simulink model "RefModel_Task"  (R2020a)
(part 3 of 5)

    |     RTInfo.Warning = ENUM_RTInfo_Warn.Warn_Path_Not_Valid;
    |     printComInfo('[System Warning] PathData Not Valid',tabspace1)
    | end
    | if ~IN_OnPlane.unlock
    | %     RTInfo.Warning = ENUM_RTInfo_Warn.Warn_SensorSystem_Not_Health;
    |     printComInfo('[System Warning] Not Unlock',tabspace1)
    | end
    | if isStallingForAWhile
    |     RTInfo.Warning = ENUM_RTInfo_Warn.Warn_Stalling;
    |     printComInfo('[System Warning] Stalling',tabspace1)
    | end
    | if ~isNaviFilterStart
    |     RTInfo.Warning = ENUM_RTInfo_Warn.Warn_FilterInit_Not_Complete;
    |     printComInfo('[System Warning] Filter Init Not Complete',tabspace1)
    | end
  function flag = isUavInFix2Rotor:
    | function flag = isUavInFix2Rotor
    | flag = false;
    | if PathModeOut.uavMode == ENUM_UAVMode.Fix2Rotor
    |     flag = true;
    | end
  function flag = isStallingForAWhile:
    | function flag = isStallingForAWhile
    | persistent lastNotStallTime stallTime0
    | if isempty(lastNotStallTime)
    |     lastNotStallTime = 0;
    |     stallTime0 = 0;
    | end
    | if ~isInStall
    |     lastNotStallTime = clock_sec; 
    | else
    |     stallTime0 = clock_sec;
    | end
    | flag = false;
    | if stallTime0 - lastNotStallTime > TaskParam.enterStallTimeSec
    |     flag = true;
    | end
  function flag = isUavInFix:
    | function flag = isUavInFix
    | flag = false;
    | if PathModeOut.uavMode == ENUM_UAVMode.Fix
    |     flag = true;
    | end
  function flag = isGetOutOfStall:
    | function flag = isGetOutOfStall
    | persistent lastStallTime notStallTime0
    | if isempty(lastStallTime)
    |     lastStallTime = 0;
    |     notStallTime0 = 0;
    | end
    | if ~isAttitudeStable_globalvar % 姿态不稳
    |     lastStallTime = clock_sec; 
    | else
    |     notStallTime0 = clock_sec;
    | end
    | flag = false;
    | if notStallTime0 - lastStallTime > 10 % 姿态稳定 10s 视为失速改出
    |     flag = true;
    | end
  function flag = willEnterManualMode:
    | function flag = willEnterManualMode
    | flag = false;
    | if ~isAutoMode_globalvar
    |     flag = true;
    | end
  function flag = willEnterAutoMode:
    | function flag = willEnterAutoMode
    | flag = false;
    | if isAutoMode_globalvar || (isNotInFense && PathModeOut.whereIsUAV == ENUM_Where.InTheAir) % && hasTaskStarted_globalbar
    |     flag = true;
    | end
  function setFlightModeInitState:
    | function setFlightModeInitState
    | % 飞机在地面的初始状态
    | PathModeOut.whereIsUAV = ENUM_Where.OnGround;  % 在地面
    | PathModeOut.uavMode = ENUM_UAVMode.Rotor;  % 旋翼
  function du_AUTO_TASK_func:
    | function du_AUTO_TASK_func
    | if isUavInRotor
    |     % dz: 固定翼航线模式下表示侧偏距，旋翼模式表示到目标点/悬停点的距离
    |     PathModeOut.distToGo = distOfTwoLL(PathModeOut.turnCenterLL(1:2),...
    |         ComFlightOut.curLLA(1:2));
    |     if all(PathModeOut.turnCenterLL(1:2)== 0) || all(ComFlightOut.curLLA(1:2)== 0)
    |         PathModeOut.distToGo = 0;
    |     end
    | end
  function sendEventWhileEnterAuto:
    | function sendEventWhileEnterAuto
    | PathModeOut.typeAutoMode = ENUM_AutoModeType.NotAutoMode; % 默认是非自动全剖面飞行
    | switch PathModeOut.whereIsUAV
    |     case ENUM_Where.OnGround % 在地面
    |         RTInfo.Task = ENUM_RTInfo_Task.Switch_AutoMode_sendEventWhileSwitchToAuto_OnGround; % 更新RT信息
    |         PathModeOut.typeAutoMode = ENUM_AutoModeType.ManualToAuto; % 只有在地面触发
    |         send(manual_groundStandBy,FLIGHTMODE.AUTO_TASK);
    |     case ENUM_Where.InTheAir % 在空中
    |         RTInfo.Task = ENUM_RTInfo_Task.Switch_AutoMode_sendEventWhileSwitchToAuto_InTheAir; % 更新RT信息
    |         isEverythingOk = ~isNotInFense && ... % 在区域内 且
    |                 PathModeOut.comStatus == ENUM_ComStatus.ComNormal; % 通信正常
    |         if isEverythingOk
    |             PathModeOut.typeAutoMode = ENUM_AutoModeType.ManualToAuto;
    |             if PathModeOut.uavMode == ENUM_UAVMode.Rotor % 空中/旋翼, 进入空中绕飞待命模式
    |                 RTInfo.Task = ENUM_RTInfo_Task.Switch_AutoMode_sendEventWhileSwitchToAuto_InTheAir_If_Rotor; % 更新RT信息
    |                 send(manual_hoverAdjust,FLIGHTMODE.AUTO_TASK);
    |             elseif PathModeOut.uavMode == ENUM_UAVMode.Fix % 空中/固定翼, 进入悬停调整模式
    |                 RTInfo.Task = ENUM_RTInfo_Task.Switch_AutoMode_sendEventWhileSwitchToAuto_InTheAir_If_Fix; % 更新RT信息
    |                 send(manual_airStandBy,FLIGHTMODE.AUTO_TASK);
    |             else
    |                 % 未处理状态
    |                 send(manual_hoverAdjust,FLIGHTMODE.AUTO_TASK);
    |                 RTInfo.Task = ENUM_RTInfo_Task.NotDefined_Fcn_sendEventWhileSwitchToAuto_If; % 更新RT信息
    |                 printComInfo('[Error] UAV is not Fix or Rotor when switch to AUTO_TASK',0)
    |             end
    |         else % 不在篱笆内 或 通信中断
    |             RTInfo.Task = ENUM_RTInfo_Task.Switch_AutoMode_sendEventWhileSwitchToAuto_InTheAir_NotInFense; % 更新RT信息
    |             printComInfo('[Info] Switch to AUTO_TASK, then enter GoHome mode',0)
    |             PathModeOut.typeAutoMode = ENUM_AutoModeType.SuspendTaskToHome;
    |             send(event_goHome_NotInFense,FLIGHTMODE.AUTO_TASK);
    |         end
    |     otherwise
    |         % 未处理状态
    |         RTInfo.Task = ENUM_RTInfo_Task.NotDefined_Fcn_sendEventWhileSwitchToAuto_Switch; % 更新RT信息
    |         printComInfo('[Error] UAV is not OnGround or InTheAir when switch to AUTO_TASK',0)
    | end
  function flag = isAllowedToEnterThisMode(mode):
    | function flag = isAllowedToEnterThisMode(mode)
    | flag = false;
    | tabspace1 = 2;
    | tabspace2 = 3;
    | % if isUavInRotor2Fix % 应对当前模式为 Rotor2Fix 或 Fix2Rotor
    | %     PathModeOut.uavMode = ENUM_UAVMode.Fix;
    | % elseif isUavInFix2Rotor
    | %     PathModeOut.uavMode = ENUM_UAVMode.Rotor;
    | % end
    | switch mode
    |     case ENUM_FlightTaskMode.TakeOffMode
    |         flag = isAllowedToTakeOff;
    |         if ~flag
    |             RTInfo.Task = ENUM_RTInfo_Task.SendEvent_TakeOff_ButNotAllowed; % 更新RT信息
    |             updateLogDataBuffer(ENUM_TaskLogBlockName.TASKLOG_FlightMode,RTInfo.Task,'write'); % 更新log缓存
    |             printComInfo('isAllowedToEnterThisMode() Switch TakeOffMode No',tabspace1)
    |             if not(isAllowedToTakeOff)
    |                 printComInfo('Not Allowed To TakeOff',tabspace2)
    |             end
    |             if ~isOnGround
    |                 printComInfo('Is Not OnGround',tabspace2)
    |             end
    |             if ~isUavInRotor
    |                 printComInfo('Is Not Rotor',tabspace2)
    |             end
    |             if not(BatteryOut.batteryStatus == ENUM_BatteryStatus.BatteryNormal)
    |                 printComInfo('BatteryLife Is Not Normal',tabspace2)
    |             end
    |         else
    |             printComInfo('isAllowedToEnterThisMode() Switch TakeOffMode Yes',tabspace1)
    |         end
    |     case ENUM_FlightTaskMode.HoverAdjustMode
    |         flag = isInTheAir && isUavInRotor && ...
    |             PathModeOut.flightTaskMode ~= ENUM_FlightTaskMode.Rotor2Fix_Mode && ...
    |             PathModeOut.flightTaskMode ~= ENUM_FlightTaskMode.Fix2Rotor_Mode;    
    |         if ~flag
    |             RTInfo.Task = ENUM_RTInfo_Task.SendEvent_HoverAdjust_ButNotAllowed; % 更新RT信息
    |             printComInfo('isAllowedToEnterThisMode() Switch HoverAdjustMode No',tabspace1)
    |             if not(isAllowedToAutoFlight)
    |                 printComInfo('Not Allowed To AutoFlight',tabspace2)
    |             end
    |             if ~isInTheAir
    |                 printComInfo('Is Not InTheAir',tabspace2)
    |             end
    |             if ~isUavInRotor
    |                 printComInfo('Is Not Rotor',tabspace2)
    |             end
    |         else
    |             printComInfo('isAllowedToEnterThisMode() Switch HoverAdjustMode Yes',tabspace1)            
    |         end
    |     case ENUM_FlightTaskMode.Rotor2Fix_Mode
    |         flag = isAllowedToAutoFlight && isInTheAir && isUavInRotor;
    |         if ~flag
    |             RTInfo.Task = ENUM_RTInfo_Task.SendEvent_Rotor2Fix_ButNotAllowed; % 更新RT信息
    |             printComInfo('isAllowedToEnterThisMode() Switch Rotor2Fix_Mode No',tabspace1)
    |             if not(isAllowedToAutoFlight)
    |                 printComInfo('Not Allowed To AutoFlight',tabspace2)
    |             end
    |             if ~isInTheAir
    |                 printComInfo('Is Not InTheAir',tabspace2)
    |             end
    |             if ~isUavInRotor
    |                 printComInfo('Is Not Rotor',tabspace2)
    |             end
    |         else
    |             printComInfo('isAllowedToEnterThisMode() Switch Rotor2Fix_Mode Yes',tabspace1)                  
    |         end
    |     case ENUM_FlightTaskMode.HoverUpMode
    |         flag = isAllowedToAutoFlight && isInTheAir && isUavInFix;
    |         if ~flag
    |             RTInfo.Task = ENUM_RTInfo_Task.SendEvent_HoverUp_ButNotAllowed; % 更新RT信息
    |             printComInfo('isAllowedToEnterThisMode() Switch HoverUpMode No',tabspace1)
    |             if not(isAllowedToAutoFlight)
    |                 printComInfo('Not Allowed To AutoFlight',tabspace2)
    |             end
    |             if ~isInTheAir
    |                 printComInfo('Is Not InTheAir',tabspace2)
    |             end
    |             if ~isUavInFix
    |                 printComInfo('Is Not Fix',tabspace2)
    |             end
    |         else
    |             printComInfo('isAllowedToEnterThisMode() Switch HoverUpMode Yes',tabspace1)                  
    |         end
    |     case ENUM_FlightTaskMode.PathFollowMode
    |         flag = isAllowedToAutoFlight && isInTheAir && isUavInFix;
    |         if ~flag
    |             RTInfo.Task = ENUM_RTInfo_Task.SendEvent_PathFollow_ButNotAllowed; % 更新RT信息
    |             printComInfo('isAllowedToEnterThisMode() Switch PathFollowMode No',tabspace1)
    |             if not(isAllowedToAutoFlight)
    |                 printComInfo('Not Allowed To AutoFlight',tabspace2)
    |             end
    |             if ~isInTheAir
    |                 printComInfo('Is Not InTheAir',tabspace2)
    |             end
    |             if ~isUavInFix
    |                 printComInfo('Is Not Fix',tabspace2)
    |             end               
    |         else
    |             printComInfo('isAllowedToEnterThisMode() Switch PathFollowMode Yes',tabspace1)                  
    |         end
    |     case ENUM_FlightTaskMode.GoHomeMode 
    |         flag = isInTheAir && (isUavInRotor || isUavInFix);
    |         if ~flag
    |             RTInfo.Task = ENUM_RTInfo_Task.SendEvent_GoHomeMode_ButNotAllowed; % 更新RT信息
    |             printComInfo('isAllowedToEnterThisMode() Switch GoHomeMode No',tabspace1)
    |             if not(isAllowedToAutoFlight)
    |                 printComInfo('Not Allowed To AutoFlight',tabspace2)
    |             end
    |             if ~isInTheAir
    |                 printComInfo('Is Not InTheAir',tabspace2)
    |             end
    |             if not(isUavInRotor || isUavInFix)
    |                 printComInfo('Is Not Fix or Rotor',tabspace2)
    |             end                  
    |         else
    |             printComInfo('isAllowedToEnterThisMode() Switch GoHomeMode Yes',tabspace1)                  
    |         end
    |     case ENUM_FlightTaskMode.HoverDownMode
    |         flag = isInTheAir && isUavInFix;
    |         if ~flag
    |             RTInfo.Task = ENUM_RTInfo_Task.SendEvent_HoverDown_ButNotAllowed; % 更新RT信息
    |             printComInfo('isAllowedToEnterThisMode() Switch HoverDownMode No',tabspace1)
    |             if not(isAllowedToAutoFlight)
    |                 printComInfo('Not Allowed To AutoFlight',tabspace2)
    |             end
    |             if ~isInTheAir
    |                 printComInfo('Is Not InTheAir',tabspace2)
    |             end
    |             if ~isUavInFix
    |                 printComInfo('Is Not Fix',tabspace2)
    |             end               
    |         else
    |             printComInfo('isAllowedToEnterThisMode() Switch HoverDownMode Yes',tabspace1)                  
    |         end
    |     case ENUM_FlightTaskMode.Fix2Rotor_Mode
    |         flag = isInTheAir && (isUavInFix || isUavInRotor2Fix);
    |         if ~flag
    |             RTInfo.Task = ENUM_RTInfo_Task.SendEvent_Fix2Rotor_ButNotAllowed; % 更新RT信息
    |             printComInfo('isAllowedToEnterThisMode() Switch Fix2Rotor_Mode No',tabspace1)
    |             if ~isInTheAir
    |                 printComInfo('Is Not InTheAir',tabspace2)
    |             end
    |             if ~isUavInFix
    |                 printComInfo('Is Not Fix',tabspace2)
    |             end                     
    |         else
    |             printComInfo('isAllowedToEnterThisMode() Switch Fix2Rotor_Mode Yes',tabspace1)                  
    |         end
    |     case ENUM_FlightTaskMode.LandMode
    |         flag = isInTheAir && isUavInRotor;
    |         if ~flag
    |             RTInfo.Task = ENUM_RTInfo_Task.SendEvent_Land_ButNotAllowed; % 更新RT信息
    |             printComInfo('isAllowedToEnterThisMode() Switch LandMode No',tabspace1)
    |             if not(isAllowedToAutoFlight)
    |                 printComInfo('Not Allowed To AutoFlight',tabspace2)
    |             end
    |             if ~isInTheAir
    |                 printComInfo('Is Not InTheAir',tabspace2)
    |             end
    |             if ~isUavInRotor
    |                 printComInfo('Is Not Rotor',tabspace2)
    |             end                 
    |         else
    |             printComInfo('isAllowedToEnterThisMode() Switch LandMode Yes',tabspace1)                  
    |         end
    |     case ENUM_FlightTaskMode.AirStandByMode
    |         flag = isInTheAir && canEnterAirStandByMode;
    |         if ~flag
    |             RTInfo.Task = ENUM_RTInfo_Task.SendEvent_AirStandBy_ButNotAllowed; % 更新RT信息
    |             printComInfo('isAllowedToEnterThisMode() Switch AirStandByMode No',tabspace1)
    |             if not(isAllowedToAutoFlight)
    |                 printComInfo('Not Allowed To AutoFlight',tabspace2)
    |             end
    |             if ~isInTheAir
    |                 printComInfo('Is Not InTheAir',tabspace2)
    |             end
    |             if not(canEnterAirStandByMode)
    |                 printComInfo('Can Not EnterAirStandByMode',tabspace2)
    |             end               
    |         else
    |             printComInfo('isAllowedToEnterThisMode() Switch AirStandByMode Yes',tabspace1)                  
    |         end
    |     otherwise
    |         RTInfo.Task = ENUM_RTInfo_Task.NotDefined_Fcn_isAllowedToEnterThisMode; % 更新RT信息
    |         printComInfo('isAllowedToEnterThisMode() Switch Otherwise',0)
    | end
  function dist = calDradiusWhileTurn(Rtarget,LL1,LL2):
    | function dist = calDradiusWhileTurn(Rtarget,LL1,LL2)
    | pos = lla2ned([LL1;0]', LL2');
    | Rnow = norm(pos(1:2));
    | dist = Rtarget - Rnow;
  function flag = isReadyToGo:
    | function flag = isReadyToGo
    | flag = 1;
    | if flag == 1 && isAttitudeStable_globalvar && isDebugInfoToShow
    |     fprintf('\t\t\t time %.2f [sec]: Ready To Go!\n',clock_sec);
    | end
  function flag = hasReachHeight(heightErr):
    | function flag = hasReachHeight(heightErr)
    | flag = false;
    | % heightErr = abs(ComFlightOut.curLLA(3)-PathModeOut.heightCmd);
    | if ComFlightOut.curLLA(3)>PathModeOut.heightCmd-heightErr
    |     flag = true;
    |     if isDebugInfoToShow
    | %         fprintf('\t\t\t time %.2f [sec]: Reach The Expected Hover Height %.0f [m]!\n',clock_sec,PathModeOut.heightCmd);
    |     end
    | end
  function headingCmd = calHeadingCmd(uavLLA_in,targetLLA_in):
    | function headingCmd = calHeadingCmd(uavLLA_in,targetLLA_in)
    | % 计算应飞航向
    | % pUAV: 无人机当前位置
    | % pointXY: 当前航线终点
    | % headingCmd: 应飞航向 (-pi,pi]
    | cPos = lla2ned(uavLLA_in, uavLLA_in(1:2));
    | target = lla2ned(targetLLA_in, uavLLA_in(1:2));
    | % 矢量
    | vec = target - cPos;
    | % 计算应飞航向
    | headingCmd = atan2(vec(2),vec(1));
  function flag = hasReachLatLon_assign(posErr):
    | function flag = hasReachLatLon_assign(posErr)
    | flag = false;
    | dLat = PathModeOut.turnCenterLL(1)- ComFlightOut.curLLA(1);
    | dLon = PathModeOut.turnCenterLL(2)- ComFlightOut.curLLA(2);
    | deg2m = 111e3;
    | dPn = dLat*deg2m;
    | dPe = dLon*deg2m*cos(ComFlightOut.curLLA(1)*pi/180);
    | dist = norm([dPn,dPe]);
    | if dist < posErr
    |     flag = true;
    | end
  function flag = isHeadingOk:
    | function flag = isHeadingOk
    | flag = false;
    | errAngle = angdiff(ComFlightOut.curEuler(1),headingCmd);
    | if abs(errAngle)<20*pi/180
    |     flag = true;
    |     printDebugInfo('AirStandBy','Already Heading To Target',2)
    | end
  function flag = isReadyToGo:
    | function flag = isReadyToGo
    | % TODO
    | flag = 1;
    | if flag == 1
    |     if isDebugInfoToShow
    |         fprintf('\t\t\t time %.2f [sec]: [HoverAdjust Mode] Ready To Go!\n',clock_sec);
    |     end
    | end
  function flag = hasReachHeight:
    | function flag = hasReachHeight
    | flag = false;
    | heightErr = abs(ComFlightOut.curLLA(3)-PathModeOut.heightCmd);
    | if ComFlightOut.curLLA(3) > PathModeOut.heightCmd - 2
    |     flag = true;
    | %     RTInfo.Task = ENUM_RTInfo_Task.If_AutoMode_HoverAdjust_ReachHeight_Yes; % 更新RT信息
    | %     if isDebugInfoToShow
    | %         fprintf('\t\t\t time %.2f [sec]: Reach The Expected Hover Height %.0f [m]!\n',clock_sec,PathModeOut.heightCmd);
    | %     end
    | end
  function flag = hasMatchAllConditons:
    | function flag = hasMatchAllConditons
    | persistent flagPre
    | if isempty(flagPre)
    |     flagPre = false;
    | end
    | flag = false;
    | if hasReachHeight && hasReachLatLon && isAttitudeStable_globalvar
    |     flag = true;
    |     RTInfo.Task = ENUM_RTInfo_Task.If_AutoMode_HoverAdjust_ReachHeightAndLevelPoint_Yes; % 更新RT信息
    |     if isDebugInfoToShow && flag ~= flagPre
    |         fprintf('\t\t\t time %.2f [sec]: Reach The Expected Hover Height %.0f [m] and Level Point (%.6f, %.6f)!\n',...
    |             clock_sec,PathModeOut.heightCmd,PathModeOut.turnCenterLL(1),PathModeOut.turnCenterLL(2));
    |     end
    | end
    | flagPre = flag;
  function flag = hasReachLatLon:
    | function flag = hasReachLatLon
    | flag = false;
    | dLat = PathModeOut.turnCenterLL(1)- ComFlightOut.curLLA(1);
    | dLon = PathModeOut.turnCenterLL(2)- ComFlightOut.curLLA(2);
    | deg2m = 111e3;
    | dPn = dLat*deg2m;
    | dPe = dLon*deg2m*cos(ComFlightOut.curLLA(1)*pi/180);
    | dist = norm([dPn,dPe]);
    | if dist < 3
    |     flag = true;
    | end
  function en_func:
    | function en_func
    | RTInfo.Task = ENUM_RTInfo_Task.Enter_AutoMode_HoverAdjust_Init; % 更新RT信息
    | updateLogDataBuffer(ENUM_TaskLogBlockName.TASKLOG_FlightMode,RTInfo.Task,'write'); % 更新log缓存
    | PathModeOut.uavMode = TaskParam.uavMode_InHoverAdjustMode;
    | PathModeOut.flightTaskMode = ENUM_FlightTaskMode.HoverAdjustMode;
    | PathModeOut.flightControlMode = ENUM_FlightControlMode.SpotHoverMode;
    | % 需计算指令： 高度 航向
    | tempIdx = idxStartPathPoint;
    | if isPathDataValid && PathModeOut.typeAutoMode == ENUM_AutoModeType.AutoProfile
    |     % 自动任务模式下
    |     printDebugInfo('HoverAdjust','Init AutoProfile Yes')
    |     RTInfo.Task = ENUM_RTInfo_Task.If_AutoMode_HoverAdjust_Init_AutoProfile_Yes; % 更新RT信息
    |     updateLogDataBuffer(ENUM_TaskLogBlockName.TASKLOG_FlightMode,RTInfo.Task,'write'); % 更新log缓存
    |     % 高度指令与前一模式相同
    |     if headingMode == 1
    |         targetLLA = double([IN_MAV.mavlink_mission_item_def(tempIdx).x,...
    |             IN_MAV.mavlink_mission_item_def(tempIdx).y, IN_MAV.mavlink_mission_item_def(tempIdx).z]);
    |         PathModeOut.headingCmd = calHeadingCmd(...
    |             ComFlightOut.curLLA,  targetLLA);
    |     else
    |         % 捕获当前航向
    |         PathModeOut.headingCmd = double(ComFlightOut.curEuler(1));
    |     end
    | else
    |     printDebugInfo('HoverAdjust','Init AutoProfile No')
    |     RTInfo.Task = ENUM_RTInfo_Task.If_AutoMode_HoverAdjust_Init_AutoProfile_No; % 更新RT信息
    |     updateLogDataBuffer(ENUM_TaskLogBlockName.TASKLOG_FlightMode,RTInfo.Task,'write'); % 更新log缓存
    |     % 捕获当前航向
    |     PathModeOut.headingCmd = double(ComFlightOut.curEuler(1));
    |     % 捕获当前高度
    |     PathModeOut.heightCmd = double(ComFlightOut.curLLA(3));
    | end
    | PathModeOut.groundspeedCmd = TaskParam.cruiseSpeed_rotorMode;
    | % 设置侧偏距为0
    | PathModeOut.dz = 0;
    | % 设置预置滚转
    | PathModeOut.rollCmd = 0;
    | % 悬停位置
    | PathModeOut.turnCenterLL = ComFlightOut.curLLA(1:2);
    | % 最大爬升率
    | PathModeOut.maxClimbSpeed = TaskParam.maxClimbSpeed_normal_TakeOffandLand;
  function responseManualMove:
    | function responseManualMove
    | persistent nFront nBack nRight nLeft
    | if isempty(nFront)
    | %     nFront = -99;
    | %     nBack = -99;
    | %     nRight = -99;
    | %     nLeft = -99;
    |     nFront = IN_MAV.mavlink_msg_arrowkey.nFront;
    |     nBack = IN_MAV.mavlink_msg_arrowkey.nBack;
    |     nRight = IN_MAV.mavlink_msg_arrowkey.nRight;
    |     nLeft = IN_MAV.mavlink_msg_arrowkey.nLeft;    
    | end
    | %%
    | nFront_cur = IN_MAV.mavlink_msg_arrowkey.nFront;
    | nBack_cur = IN_MAV.mavlink_msg_arrowkey.nBack;
    | nRight_cur = IN_MAV.mavlink_msg_arrowkey.nRight;
    | nLeft_cur = IN_MAV.mavlink_msg_arrowkey.nLeft;
    | distFront = IN_MAV.mavlink_msg_arrowkey.distFront;
    | distRight = IN_MAV.mavlink_msg_arrowkey.distRight;
    | distBack = IN_MAV.mavlink_msg_arrowkey.distBack;
    | distLeft = IN_MAV.mavlink_msg_arrowkey.distLeft;
    | curLat = ComFlightOut.curLLA(1);
    | %%
    | dP_lat = 0;
    | dP_lon = 0;
    | heading = ComFlightOut.curEuler(1);
    | if nFront ~= nFront_cur
    |     angle = heading + 0;
    |     dP_lat = dP_lat + distFront*cos(angle);
    |     dP_lon = dP_lon + distFront*sin(angle);
    |     RTInfo.Task = ENUM_RTInfo_Task.Event_GSKeyMove_North;
    |     printComInfo('Key Move: Front %.0fm',1,distFront);
    | end
    | if nBack ~= nBack_cur
    |     angle = heading + pi;
    |     dP_lat = dP_lat + distBack*cos(angle);
    |     dP_lon = dP_lon + distBack*sin(angle);
    |     RTInfo.Task = ENUM_RTInfo_Task.Event_GSKeyMove_South;
    |     printComInfo('Key Move: Back %.0fm',1,distBack);
    | end
    | if nRight ~= nRight_cur
    |     angle = heading + pi/2;
    |     dP_lat = dP_lat + distRight*cos(angle);
    |     dP_lon = dP_lon + distRight*sin(angle);
    |     RTInfo.Task = ENUM_RTInfo_Task.Event_GSKeyMove_East;
    |     printComInfo('Key Move: Right %.0fm',1,distRight);
    | end
    | if nLeft ~= nLeft_cur
    |     angle = heading + 3/2*pi;
    |     dP_lat = dP_lat + distLeft*cos(angle);
    |     dP_lon = dP_lon + distLeft*sin(angle);
    |     RTInfo.Task = ENUM_RTInfo_Task.Event_GSKeyMove_West;
    |     printComInfo('Key Move: Left %.0fm',1,distLeft);
    | end
    | nFront = IN_MAV.mavlink_msg_arrowkey.nFront;
    | nBack = IN_MAV.mavlink_msg_arrowkey.nBack;
    | nRight = IN_MAV.mavlink_msg_arrowkey.nRight;
    | nLeft = IN_MAV.mavlink_msg_arrowkey.nLeft;
    | 
    | dlat_deg = m2lat(dP_lat);
    | dlon_deg = m2lon(dP_lon,curLat);
    | if dlat_deg ~= 0 || dlon_deg ~= 0
    |     PathModeOut.turnCenterLL = PathModeOut.turnCenterLL + [dlat_deg,dlon_deg];
    |     ComFlightOut.curHomeLLA(1:2) = PathModeOut.turnCenterLL;
    |     RTInfo.Task = ENUM_RTInfo_Task.TaskLog_Input_HomeChange_KeyBoard;% 更新RTInfo Task
    |     updateLogDataBuffer(ENUM_TaskLogBlockName.TASKLOG_ParserInput,RTInfo.Task,'write'); % 更新log缓存
    | end
  function en_func:
    | function en_func
    | printDebugInfo('HoverAdjust','Doing')
    | RTInfo.Task = ENUM_RTInfo_Task.Enter_AutoMode_HoverAdjust_Doing; % 更新RT信息
    | updateLogDataBuffer(ENUM_TaskLogBlockName.TASKLOG_FlightMode,RTInfo.Task,'write'); % 更新log缓存
    | switch PathModeOut.typeAutoMode
    |     case ENUM_AutoModeType.SuspendTaskToHomeThenLand
    |         printDebugInfo('HoverAdjust','Switch SuspendTaskToHomeThenLand')
    |         RTInfo.Task = ENUM_RTInfo_Task.Switch_AutoMode_HoverAdjust_Doing_SuspendTaskToHome; % 更新RT信息
    |         updateLogDataBuffer(ENUM_TaskLogBlockName.TASKLOG_FlightMode,RTInfo.Task,'write'); % 更新log缓存
    |         PathModeOut.turnCenterLL = ComFlightOut.curHomeLLA(1:2);
    |     case  ENUM_AutoModeType.SuspendTaskToLand
    |         printDebugInfo('HoverAdjust','Switch SuspendTaskToLand')
    |         RTInfo.Task = ENUM_RTInfo_Task.Switch_AutoMode_HoverAdjust_Doing_SuspendTaskToLand; % 更新RT信息
    |         updateLogDataBuffer(ENUM_TaskLogBlockName.TASKLOG_FlightMode,RTInfo.Task,'write'); % 更新log缓存
    |         if landPosMode == ENUM_LandMode.HomeVTL
    |             PathModeOut.turnCenterLL = ComFlightOut.curHomeLLA(1:2);
    |         else
    |             PathModeOut.turnCenterLL = ComFlightOut.curLLA(1:2);
    |         end
    |     case ENUM_AutoModeType.SuspendTaskToHome
    |         printDebugInfo('HoverAdjust','Switch SuspendTaskToHome')
    |         RTInfo.Task = ENUM_RTInfo_Task.Switch_AutoMode_HoverAdjust_Doing_SuspendTaskToHome; % 更新RT信息
    |         updateLogDataBuffer(ENUM_TaskLogBlockName.TASKLOG_FlightMode,RTInfo.Task,'write'); % 更新log缓存
    |         PathModeOut.turnCenterLL = ComFlightOut.curLLA(1:2);
    |     case ENUM_AutoModeType.Fix2Rotor2HoverAdjust
    |         printDebugInfo('HoverAdjust','Switch Fix2Rotor2HoverAdjust')
    |         RTInfo.Task = ENUM_RTInfo_Task.Switch_AutoMode_HoverAdjust_Doing_Fix2Rotor2HoverAdjust; % 更新RT信息
    |         updateLogDataBuffer(ENUM_TaskLogBlockName.TASKLOG_FlightMode,RTInfo.Task,'write'); % 更新log缓存
    |         PathModeOut.turnCenterLL = ComFlightOut.curLLA(1:2);
    |     case ENUM_AutoModeType.AutoProfile
    |         printDebugInfo('HoverAdjust','Switch AutoProfile')
    |         RTInfo.Task = ENUM_RTInfo_Task.Switch_AutoMode_HoverAdjust_Doing_AutoProfile; % 更新RT信息
    |         updateLogDataBuffer(ENUM_TaskLogBlockName.TASKLOG_FlightMode,RTInfo.Task,'write'); % 更新log缓存
    |         if nextMode == ENUM_FlightTaskMode.LandMode
    |             PathModeOut.turnCenterLL = ComFlightOut.curHomeLLA(1:2);
    |         end
    |     case ENUM_AutoModeType.PauseInAir
    |         RTInfo.Task = ENUM_RTInfo_Task.Switch_AutoMode_HoverAdjust_Doing_PauseInAir; % 更新RT信息
    |         updateLogDataBuffer(ENUM_TaskLogBlockName.TASKLOG_FlightMode,RTInfo.Task,'write'); % 更新log缓存        
    |         PathModeOut.typeAutoMode = typeAutoModePre;
    |         send(event_gotoWaitForContinue,FLIGHTMODE.AUTO_TASK)
    |     case ENUM_AutoModeType.Fix2Rotor2Home2Land
    |         printDebugInfo('HoverAdjust','Switch Fix2Rotor2Home2Land')
    |         RTInfo.Task = ENUM_RTInfo_Task.Switch_AutoMode_HoverAdjust_Doing_PauseInAir; % 更新RT信息
    |         updateLogDataBuffer(ENUM_TaskLogBlockName.TASKLOG_FlightMode,RTInfo.Task,'write'); % 更新log缓存              
    |         PathModeOut.turnCenterLL = ComFlightOut.curHomeLLA(1:2);
    |     otherwise
    |         % printDebugInfo('HoverAdjust','Switch Otherwise')
    |         RTInfo.Task = ENUM_RTInfo_Task.Switch_AutoMode_HoverAdjust_Doing_Otherwise; % 更新RT信息
    |         updateLogDataBuffer(ENUM_TaskLogBlockName.TASKLOG_FlightMode,RTInfo.Task,'write'); % 更新log缓存             
    |         RTInfo.Task = ENUM_RTInfo_Task.NotDefined_State_HoverAdjust_Doing_Switch; % 更新RT信息
    | end
  function dHeading = calHeadingErr(headingCmd,headingNow):
    | function dHeading = calHeadingErr(headingCmd,headingNow)
    | % 计算飞机当前航向偏差
    | % headingCmd: 指令航向 rad
    | % headingNow：当前航向 rad
    | % dHeading: 航向差 rad
    | headingNow = rem(headingNow,2*pi);
    | headingCmd = rem(headingCmd,2*pi);
    | sub = zeros(3,1);
    | psi_d_possible = zeros(3,1);
    | psi_d_possible(1) = headingCmd;
    | psi_d_possible(2) = headingCmd-2*pi;
    | psi_d_possible(3) = headingCmd+2*pi;
    | sub(1) = psi_d_possible(1)-headingNow;
    | sub(2) = psi_d_possible(2)-headingNow;
    | sub(3) = psi_d_possible(3)-headingNow;
    | [~,ind] = min(abs(sub));
    | dHeading = sub(ind);
    | 
    | % % 测试用例
    | % if 0
    | %     headingCmd = 181*pi/180;
    | %     headingNow = 179*pi/180;
    | %     dHeading = calHeadingErr(headingCmd,headingNow)*180/pi
    | %     
    | %     headingCmd = 361*pi/180;
    | %     headingNow = 359*pi/180;    
    | %     dHeading = calHeadingErr(headingCmd,headingNow)*180/pi    
    | %     
    | %     
    | %     headingCmd = -361*pi/180;
    | %     headingNow = -359*pi/180;
    | %     dHeading = calHeadingErr(headingCmd,headingNow)*180/pi  
    | %     
    | %     headingCmd = -1*pi/180;
    | %     headingNow = 0*pi/180;
    | %     dHeading = calHeadingErr(headingCmd,headingNow)*180/pi      
    | %     
    | %     headingCmd = -181*pi/180;
    | %     headingNow = 180*pi/180;
    | %     dHeading = calHeadingErr(headingCmd,headingNow)*180/pi    
    | % end
  function flag = hasReachExpectSpeed(airspeed_req,groundspeed_req):
    | function flag = hasReachExpectSpeed(airspeed_req,groundspeed_req)
    | flag = false;
    | if ComFlightOut.curGroundSpeed > groundspeed_req && ComFlightOut.curAirSpeed > airspeed_req
    |     flag = true;
    |     RTInfo.Task = ENUM_RTInfo_Task.If_AutoMode_Rotor2Fix_ReachSpeed_Yes; % 更新RT信息
    |     if isDebugInfoToShow
    | %         fprintf('\t\t\t time %.2f [sec]: Reach Expected Speed!\n',clock_sec);
    |     end
    | end
  function flag = calIfReachPoint_horizontal(uavLLA,point1LLA,point2LLA,In_AlgoParams):
    | function flag = calIfReachPoint_horizontal(uavLLA,point1LLA,point2LLA,In_AlgoParams)
    | % 判断是否到达目标点
    | % uavLLA: 当前位置
    | % point1LLA：航段起点位置
    | % point2LLA：航段终点位置
    | % In_AlgoParams: 参数
    | pUAV = lla2ned(uavLLA, uavLLA(1:2));
    | point1XY = lla2ned(point1LLA, uavLLA(1:2));
    | point2XY = lla2ned(point2LLA, uavLLA(1:2));
    | pUAV(3) = 0;
    | point1XY(3) = 0;
    | point2XY(3) = 0;
    | mode = In_AlgoParams.reachDetermineMode;
    | flag = false;
    | switch mode
    |     case 0 %
    |         reachFlag_point = calPointModeFlag(pUAV,point2XY,In_AlgoParams.reachFlag_point_dist);
    |         flag = reachFlag_point;
    |     case 1 %
    |         reachFlag_line = calLineModeFlag(pUAV,point2XY,point1XY,In_AlgoParams.reachFlag_line_dist);
    |         flag = reachFlag_line;
    |     case 2 %
    |         reachFlag_point = calPointModeFlag(pUAV,point2XY,In_AlgoParams.reachFlag_point_dist);
    |         reachFlag_line = calLineModeFlag(pUAV,point2XY,point1XY,In_AlgoParams.reachFlag_line_dist);
    |         flag = reachFlag_point | reachFlag_line;
    |     otherwise
    |         RTInfo.Task = ENUM_RTInfo_Task.NotDefined_Fcn_calIfReachPoint_Switch; % 更新RT信息
    |         error('Wrong set!')
    | end
    | if flag
    |      sl = 1; 
    | end
    | %% 点距判定
    | function reachFlag = calPointModeFlag(pUAV,point2XY,reachFlag_point_dist)
    | reachFlag = false;
    | dist = norm(pUAV-point2XY);
    | if dist <= reachFlag_point_dist
    |     reachFlag = true;
    | end
    | % test
    | if dist < 10
    |     test = 1; 
    | end
    | %% 过线判定
    | function reachFlag = calLineModeFlag(pUAV,point2XY,point1XY,reachFlag_point_dist)
    | vec1 = pUAV-point1XY;
    | vec2 = point2XY-point1XY;
    | len1 = norm(vec1);
    | len2 = norm(vec2);
    | if len1 == 0 || len2 == 0
    |     angle = 0;
    | else
    |     % 真的出现过acos(1.000000000000001)产生复数
    |     temp = dot(vec1,vec2)/(len1*len2+eps);
    |     if temp > 1
    |         temp = 1;
    |     elseif temp < -1
    |         temp = -1;
    |     end
    |     angle = acos(temp);
    | end
    | reachFlag = false;
    | if (abs(len1*cos(angle)) > len2 - reachFlag_point_dist) && abs(angle)<pi/2
    |     reachFlag = true;
    | end
    | if len1*cos(angle)-len2 < 10
    |     test = 1; 
    | end
  function out = calEnterLLToFlyAround(centerLL,curLL,R):
    | function out = calEnterLLToFlyAround(centerLL,curLL,R)
    | % out;目标[纬度，精度]deg
    | % centerLL: home点[纬度，精度]deg，作为绕飞圆心
    | % curLL：起始位置
    | % R: 盘旋半径
    | [tangencyLL1,tangencyLL2] = findTangencyPointsLLA(centerLL,curLL,R);
    | mode = 'clockwise'; % anticlockwise
    | switch mode
    |     case 'clockwise'
    |         out = tangencyLL1;
    |     otherwise
    |         out = tangencyLL2;
    | end
  function en_func_HoverUp:
    | function en_func_HoverUp
    | % 需计算指令： 高度 速度 滚转角 转弯半径
    | tempIdx = 1; % 使用home点的高度  idxStartPathPoint;
    | PathModeOut.turnRadiusCmd = TaskParam.turnR;
    | if isPathDataValid && PathModeOut.typeAutoMode == ENUM_AutoModeType.AutoProfile
    |     RTInfo.Task = ENUM_RTInfo_Task.If_AutoMode_HoverUp_Init_AutoProfile_Yes; % 更新RT信息
    |     updateLogDataBuffer(ENUM_TaskLogBlockName.TASKLOG_FlightMode,RTInfo.Task,'write'); % 更新log缓存    
    |     PathModeOut.heightCmd = double(ComFlightOut.curLLA(3));
    |     PathModeOut.groundspeedCmd = TaskParam.cruiseSpeed_cruise;
    | else % 手动选择该模式
    |     % 捕获当前高度
    |     PathModeOut.heightCmd = double(ComFlightOut.curLLA(3));
    |     % 捕获当前速度,设定最小值
    |     PathModeOut.groundspeedCmd = max(TaskParam.cruiseSpeed_cruise,ComFlightOut.curGroundSpeed);
    | end
    | % PathModeOut.turnRadiusCmd = AlgoParams.turnR;
    | PathModeOut.rollCmd = ...
    |     atan(PathModeOut.groundspeedCmd^2/PathModeOut.turnRadiusCmd/9.8);
    | 
    | % 设置侧偏距为0
    | PathModeOut.dz = 0;
    | % 绕飞中心
    | if preTaskMode ~= ENUM_FlightTaskMode.HoverUpMode && ...
    |         preTaskMode ~= ENUM_FlightTaskMode.HoverDownMode
    |     % 距离home点距离
    |     distToHome = distOfTwoLL(ComFlightOut.curHomeLLA(1:2)', ComFlightOut.curLLA(1:2));
    |     if ~TaskParam.isHoverUpDownWithHome || distToHome > 300 
    |         % 当不以home点为盘旋中心，或当前位置距离home过远时
    |         [dLat,dLon] = calDLatLonOfRotateCenterFromCurPos(...
    |             ComFlightOut.curLLA(1:2)',ComFlightOut.curEuler(1),PathModeOut.turnRadiusCmd,'right');
    |         PathModeOut.turnCenterLL =  ComFlightOut.curLLA(1:2) + [dLat,dLon];
    |     else
    |         % 以home点为盘旋中心，且home点在附近
    |         PathModeOut.turnCenterLL =  ComFlightOut.curHomeLLA(1:2);
    |         RTInfo.Task = ENUM_RTInfo_Task.If_AutoMode_INIT_CircleHome; % 更新RT信息
    |         updateLogDataBuffer(ENUM_TaskLogBlockName.TASKLOG_FlightMode,RTInfo.Task,'write'); % 更新log缓存
    |     end
    | else
    |     % 沿用HoverUpDown模式的，确保盘旋中心一致
    |     RTInfo.Task = ENUM_RTInfo_Task.HoverUp_INIT_ContinueHoverUpDown; % 更新RT信息
    |     updateLogDataBuffer(ENUM_TaskLogBlockName.TASKLOG_FlightMode,RTInfo.Task,'write'); % 更新log缓存
    | end
    | % 最大爬升率
    | PathModeOut.maxClimbSpeed = TaskParam.maxClimbSpeed_fixMode + 0.7;
  function flag = hasReachExpectedHeight:
    | function flag = hasReachExpectedHeight
    | flag = false;
    | if ComFlightOut.curLLA(3) > PathModeOut.heightCmd - 10
    |     flag = true;
    | %     RTInfo.Task = ENUM_RTInfo_Task.If_AutoMode_HoverUp_ReachHeight_Yes; % 更新RT信息
    | %     if isDebugInfoToShow
    | %         fprintf('\t\t\t time %.2f [sec]: Reach The Expected Hover Height %.0f [m]!\n',clock_sec,PathModeOut.heightCmd);
    | %     end
    | end
  function flag = hasReachExpectedHeightRange:
    | function flag = hasReachExpectedHeightRange
    | flag = false;
    | heightErr = abs(ComFlightOut.curLLA(3)-PathModeOut.heightCmd);
    | range = 10;
    | if heightErr < range
    |     flag = true;
    |     RTInfo.Task = ENUM_RTInfo_Task.If_AutoMode_HoverUp_ReachHeightRange_Yes; % 更新RT信息
    |     if isDebugInfoToShow
    |         fprintf('\t\t\t time %.2f [sec]: Reach The Expected Hover Height Range, Current Height is %.0f [m]!\n',clock_sec,PathModeOut.heightCmd);
    |     end
    | end
  function en_func_HoverUp_SingleMode:
    | function en_func_HoverUp_SingleMode
    | % 需计算指令： 高度 速度 滚转角 转弯半径
    | PathModeOut.turnRadiusCmd = TaskParam.turnR;
    | PathModeOut.heightCmd = double(ComFlightOut.curLLA(3)) + 100;
    | PathModeOut.groundspeedCmd = TaskParam.cruiseSpeed_cruise;
    | PathModeOut.rollCmd = ...
    |     atan(PathModeOut.groundspeedCmd^2/PathModeOut.turnRadiusCmd/9.8);
    | % 设置侧偏距为0
    | PathModeOut.dz = 0;
    | % 绕飞中心
    | [dLat,dLon] = calDLatLonOfRotateCenterFromCurPos(...
    |     ComFlightOut.curLLA(1:2)',ComFlightOut.curEuler(1),PathModeOut.turnRadiusCmd,'right');
    | PathModeOut.turnCenterLL =  ComFlightOut.curLLA(1:2) + [dLat,dLon];
    | % 最大爬升率
    | PathModeOut.maxClimbSpeed = TaskParam.maxClimbSpeed_fixMode;
  function updateTurnR_HoverUp:
    | function updateTurnR_HoverUp
    | % du_func_HoverUp_Doing
    | if ComFlightOut.curLLA(3) > TaskParam.beginHeight_expandRadiusInHoverUp
    |     % 半径扩张 (可以省电，但注意高度阈值的选择不易过低，否则有碰撞风险)
    |     dh = abs(ComFlightOut.curLLA(3) - TaskParam.beginHeight_expandRadiusInHoverUp);
    |     PathModeOut.turnRadiusCmd = TaskParam.turnR + TaskParam.k_expandRadiusInHoverUp*dh;
    |     PathModeOut.turnRadiusCmd = min(PathModeOut.turnRadiusCmd,TaskParam.maxRadiusInHoverUp);
    | end
    | PathModeOut.turnRadiusCmd_HoverUp = PathModeOut.turnRadiusCmd;
    | PathModeOut.dR_turn = calDradiusWhileTurn(PathModeOut.turnRadiusCmd,...
    |     ComFlightOut.curLLA(1:2)',PathModeOut.turnCenterLL);
  function flag = isHeadingToTarget:
    | function flag = isHeadingToTarget
    | flag = false;
    | tempIdx = idxStartPathPoint;
    | targetLLA = double([IN_MAV.mavlink_mission_item_def(tempIdx).x,...
    |     IN_MAV.mavlink_mission_item_def(tempIdx).y, IN_MAV.mavlink_mission_item_def(tempIdx).z]);
    | headingCmd = calHeadingCmd(ComFlightOut.curLLA,  targetLLA);
    | errAngle = angdiff(ComFlightOut.curEuler(1),headingCmd);
    | 
    | dist = distOfTwoLL(targetLLA(1:2),ComFlightOut.curLLA(1:2));
    | if abs(errAngle)<25*pi/180 || dist < 160
    |     flag = true;
    |     printDebugInfo('AirStandBy','Already Heading To Target',2)
    | end
  function record1(value):
    | function record1(value)
    | % record1
    | if value >= 90 && value < 120
    |     printDebugInfo('HoverUp','Expand R >= 90')
    | elseif value >= 120
    |     printDebugInfo('HoverUp','Expand R >= 120')
    | end
    | RTInfo.Task = ENUM_RTInfo_Task.HoverUp_Expand_R; % 更新RT信息
    | updateLogDataBuffer(ENUM_TaskLogBlockName.TASKLOG_FlightMode,RTInfo.Task,'write',[PathModeOut.turnRadiusCmd;0;0;0;0]); % 更新log缓存
  function SendEvent_autoGoToNextMode:
    | function SendEvent_autoGoToNextMode
    | send(auto_gotoNextMode,FLIGHTMODE.AUTO_TASK)
  function updateLLATaksInterrupt:
    | function updateLLATaksInterrupt
    | PathModeOut.LLATaskInterrupt = [...
    |     ComFlightOut.curLLA(1);...
    |     ComFlightOut.curLLA(2);...
    |     PathModeOut.heightCmd;];
    | PathModeOut.lastTargetPathPoint = PathModeOut.currentPointNum;
  function PathModeOut_out  = updatePathModeStruct(curLLA_param,startLLA_param,targetLLA_param,PathModeOut_in,mission_item_def_param):
    | function PathModeOut_out  = updatePathModeStruct(curLLA_param,startLLA_param,targetLLA_param,PathModeOut_in,mission_item_def_param)
    | % 更新航线模式的输出参数
    | PathModeOut_out = PathModeOut_in;
    | % 计算应飞航向
    | PathModeOut_out.headingCmd = calHeadingCmd(...
    |     curLLA_param,targetLLA_param);
    | % 计算剩余距离
    | PathModeOut_out.distToGo = calPointDist_horizontal(...
    |     curLLA_param, targetLLA_param);
    | % 计算侧偏距
    | PathModeOut_out.dz = calDz(ComFlightOut.curLLA,  ...
    |     startLLA_param,targetLLA_param);
    | % % 计算指令速度
    | % PathModeOut_out.groundspeedCmd = double(mission_item_def_param.param4);
    | % 计算转弯半径
    | % PathModeOut_out.turnRadiusCmd = 0;
    | % 计算指令高度
    | PathModeOut_out.heightCmd = double(mission_item_def_param.z);
  function updateTaskCompleteFlag:
    | function updateTaskCompleteFlag
    | PathModeOut.isTaskComplete = true;
  function dz = calDz(uavLLA,point1LLA,point2LLA):
    | function dz = calDz(uavLLA,point1LLA,point2LLA)
    | % 计算飞机当前位置偏离航线的距离
    | % pUAV: 无人机当前位置
    | % point0：当前航线起点
    | % point1: 当前航线终点
    | % dz: 侧偏距，从天顶俯视，飞机在航线右侧偏距为正
    | pUAV = lla2ned(uavLLA, point2LLA(1:2));
    | point1XY = lla2ned(point1LLA, point2LLA(1:2));
    | point2XY = lla2ned(point2LLA, point2LLA(1:2));
    | cPos = [pUAV(1:2),0];
    | point1 = [point1XY(1:2),0];
    | point2 = [point2XY(1:2),0];
    | % 矢量
    | vec1 = cPos-point1;
    | vec2 = point2-point1;
    | len1 = norm(vec1);
    | len2 = norm(vec2);
    | z = cross(vec1,vec2);
    | % 侧偏距
    | dz_sign = sign(z(3));
    | if len1 == 0 || len2 == 0
    |     sin_angle = 0;
    | else
    |     sin_angle = abs(norm(z)/len1/len2);
    | end
    | if abs(sin_angle) <= 1+1e-5
    |     sin_angle = min(max(sin_angle,-1),1);
    | elseif abs(sin_angle) > 1+1e-5
    |     sin_angle = sign(sin_angle);
    |     filename = 'calDz';
    |     error(['A error happened in ',filename]);
    | end
    | angle = asin(sin_angle);
    | dz = dz_sign*abs(sin(angle)*len1);
    | if isnan(dz)
    |     sl = 1;
    | end
    | %% 测试用例：
    | % if 0
    | %     num = 20;
    | %     point1XY = [-1,-1];
    | %     point2XY = [1,1];
    | %     figure(112)
    | %     plot(point1XY(1),point1XY(2),'ro');hold on;
    | %     plot(point2XY(1),point2XY(2),'bo');hold on;
    | %     plot([point1XY(1),point2XY(1)],[point1XY(2),point2XY(2)]);hold on;
    | %     grid on;
    | %     axis equal
    | %     xlim([-3,3])
    | %     ylim([-3,3])
    | %     pUAV = 1*randn(num,2);
    | %     for i = 1:num
    | %         dz(i) = calDz(pUAV(i,:),point1XY,point2XY);
    | %         plot(pUAV(i,1),pUAV(i,2),'k*');hold on;
    | %         text(pUAV(i,1)+0.2,pUAV(i,2)+0.2,[num2str(dz(i))]);hold on;
    | %     end
    | % end
  function flag = isNextTheLastPoint:
    | function flag = isNextTheLastPoint
    | % 计算有效航点数
    | flag = 0;
    | if PathModeOut.currentPointNum == PathModeOut.validPathNum
    |     flag = 1;
    | end
  function calTransitPoints:
    | function calTransitPoints
    | testflag = isAddTransitPoint && TaskParam.isInterpPathPoints;
    | % 判断当前航点和前置航点的距离
    | tempIdx = PathModeOut.prePointNum;
    | prePathLLA = double([IN_MAV.mavlink_mission_item_def(tempIdx).x,...
    |     IN_MAV.mavlink_mission_item_def(tempIdx).y, IN_MAV.mavlink_mission_item_def(tempIdx).z]);
    | tempIdx = PathModeOut.currentPointNum;
    | curPathLLA = double([IN_MAV.mavlink_mission_item_def(tempIdx).x,...
    |     IN_MAV.mavlink_mission_item_def(tempIdx).y, IN_MAV.mavlink_mission_item_def(tempIdx).z]);
    | distFromPrepathpointToCurpathpoint = distOfTwoLL(curPathLLA(1:2),prePathLLA(1:2));
    | if distFromPrepathpointToCurpathpoint < 1
    |     testflag = false;
    | end
    | % testflag = false;
    | if ~testflag
    |     % 航段起点
    |     tempIdx = PathModeOut.prePointNum;
    |     startLLA = double([IN_MAV.mavlink_mission_item_def(tempIdx).x,...
    |         IN_MAV.mavlink_mission_item_def(tempIdx).y, IN_MAV.mavlink_mission_item_def(tempIdx).z]);
    |     % 航段终点
    |     tempIdx = PathModeOut.currentPointNum;
    |     targetLLA = double([IN_MAV.mavlink_mission_item_def(tempIdx).x,...
    |         IN_MAV.mavlink_mission_item_def(tempIdx).y, IN_MAV.mavlink_mission_item_def(tempIdx).z]);
    |     
    |     temp_AlgoParams = TaskParam;
    |     kk = ComFlightOut.curGroundSpeed/(TaskParam.cruiseSpeed_cruise+eps);
    |     if isnan(kk)
    |         kk = 1;
    |     end
    |     kk = min(1.2,kk);
    |     kk = max(0.8,kk);
    |     temp_AlgoParams.reachFlag_point_dist = kk*temp_AlgoParams.reachFlag_point_dist; 
    |     arriveFlag = calIfReachPoint_horizontal(ComFlightOut.curLLA,  ...
    |         startLLA,  targetLLA,  temp_AlgoParams);
    | else
    |     minPoint0 = zeros(1,3);
    |     minPoint1 = zeros(1,3);
    |     minPoint2 = zeros(1,3);
    |     if PathModeOut.currentPointNum <= 2
    |         PathModeOut.currentPointNum = 3;
    |     end
    |     tempIdx = PathModeOut.currentPointNum-2;
    |     prepreLLA = double([IN_MAV.mavlink_mission_item_def(tempIdx).x,...
    |         IN_MAV.mavlink_mission_item_def(tempIdx).y, IN_MAV.mavlink_mission_item_def(tempIdx).z]);
    |     tempIdx = PathModeOut.currentPointNum-2;
    |     prepreLLA = double([IN_MAV.mavlink_mission_item_def(tempIdx).x,...
    |         IN_MAV.mavlink_mission_item_def(tempIdx).y, IN_MAV.mavlink_mission_item_def(tempIdx).z]);
    |     tempIdx = PathModeOut.currentPointNum-1;
    |     preLLA = double([IN_MAV.mavlink_mission_item_def(tempIdx).x,...
    |         IN_MAV.mavlink_mission_item_def(tempIdx).y, IN_MAV.mavlink_mission_item_def(tempIdx).z]);
    |     tempIdx = PathModeOut.currentPointNum;
    |     curLLA = double([IN_MAV.mavlink_mission_item_def(tempIdx).x,...
    |         IN_MAV.mavlink_mission_item_def(tempIdx).y, IN_MAV.mavlink_mission_item_def(tempIdx).z]);
    |     tempIdx = PathModeOut.currentPointNum+1;
    |     nextLLA = double([IN_MAV.mavlink_mission_item_def(tempIdx).x,...
    |         IN_MAV.mavlink_mission_item_def(tempIdx).y, IN_MAV.mavlink_mission_item_def(tempIdx).z]);
    |     minPoint0(3) = curLLA(3);
    |     minPoint1(3) = curLLA(3);
    |     minPoint2(3) = curLLA(3);
    |     curXY = lla2ned(curLLA,preLLA(1:2));
    |     curLen = norm(curXY(1:2));
    |       
    |     pathspace = max(20,min(curLen/2.5,50));
    |     pathangle = 30*pi/180;
    |     
    |     preTaskPathHeading = calPathHeading(preLLA(1:2),prepreLLA(1:2));
    |     curPathHeading = calPathHeading(curLLA(1:2),preLLA(1:2));
    |     nextTaskPathHeading = calPathHeading(nextLLA(1:2),curLLA(1:2));
    |     
    |     headingErr = abs(angdiff(preTaskPathHeading,nextTaskPathHeading));
    |     % 第0个点
    |     R = rotZ(nextTaskPathHeading);
    |     midPos = R'*[20;0;0];
    |     deg2m = 6378e3*2*pi/360;
    |     dLon = 1/deg2m*midPos(2)/cos(curLLA(1)*pi/180);
    |     dLat = 1/deg2m*midPos(1);
    |     minPoint0(1) = curLLA(1) - dLat;
    |     minPoint0(2) = curLLA(2) - dLon;    
    |     % 第一个点
    |     addangle = pathangle*sign(-angdiff(curPathHeading,nextTaskPathHeading));
    |     nextTaskPathHeading = nextTaskPathHeading + 1*addangle;
    |     R = rotZ(nextTaskPathHeading);
    |     midPos = R'*[pathspace;0;0];
    |     deg2m = 6378e3*2*pi/360;
    |     dLon = 1/deg2m*midPos(2)/cos(curLLA(1)*pi/180);
    |     dLat = 1/deg2m*midPos(1);
    |     minPoint1(1) = minPoint0(1) - dLat;
    |     minPoint1(2) = minPoint0(2) - dLon;
    |     % 第二个点
    |     nextTaskPathHeading = nextTaskPathHeading + 2*addangle;
    |     R = rotZ(nextTaskPathHeading);
    |     midPos = R'*[pathspace;0;0];
    |     deg2m = 6378e3*2*pi/360;
    |     dLon = 1/deg2m*midPos(2)/cos(curLLA(1)*pi/180);
    |     dLat = 1/deg2m*midPos(1);
    |     minPoint2(1) = minPoint1(1) - dLat;
    |     minPoint2(2) = minPoint1(2) - dLon;
    |     if idxTransitPoint == 0
    |         % 航段起点
    |         startLLA = preLLA;
    |         % 航段终点
    |         targetLLA = minPoint2;
    |     elseif idxTransitPoint == 1
    |         % 航段起点
    |         startLLA = minPoint2;
    |         % 航段终点
    |         targetLLA = minPoint1;  
    |     elseif idxTransitPoint == 2
    |         % 航段起点
    |         startLLA = minPoint1;
    |         % 航段终点
    |         targetLLA = minPoint0;        
    |     else
    |         % 航段起点
    |         startLLA = minPoint0;
    |         % 航段终点
    |         targetLLA = curLLA;
    |     end
    |     temp_AlgoParams = TaskParam;
    |     arriveTransitPointFlag = calIfReachPoint_horizontal(ComFlightOut.curLLA,  ...
    |         startLLA,  targetLLA,  temp_AlgoParams);
    |     arriveFlag = false;
    |     if arriveTransitPointFlag
    |         if idxTransitPoint < 4
    |             idxTransitPoint = idxTransitPoint + 1;
    |         end
    |         if idxTransitPoint == 4
    |             arriveFlag = true;
    |         end
    |     end
    | end
    | PathModeOut.prePathPoint_LLA = startLLA;
    | PathModeOut.curPathPoint_LLA = targetLLA;
    | % 更新PathMode输出结构体
    | this_mission_item_def = IN_MAV.mavlink_mission_item_def(tempIdx);
    | PathModeOut  = updatePathModeStruct(ComFlightOut.curLLA,...
    |     startLLA,  targetLLA,  PathModeOut,  this_mission_item_def);
    | 
    | if (testflag && idxTransitPoint == 0) || ...
    |         isAddTransitPoint || ...
    |         (~testflag && IN_MAV.mavlink_mission_item_def(PathModeOut.currentPointNum).param1 == 0)
    |     PathModeOut.dz = 0;
    | end
    | 
    | function R = rotZ(yaw)
    | R = [cos(yaw) sin(yaw) 0;
    |     -sin(yaw) cos(yaw) 0;
    |     0        0        1;];
    | 
    | function angle = calPathHeading(LLt,LL0)
    | lla = [LLt,0];
    | pos = lla2ned(lla, LL0);
    | angle = atan2(pos(2),pos(1));
    | 
    | % function flag = isAddTransitPoint
    | % flag = false;
    | % if isArrive1stPointInPathMode && ... 表示是否已经进入航线（已经到达第一个点）
    | %         mission_item_def(tempIdx).param1 == 0 && ... 该航段为非任务航段（不拍照）
    | %         PathModeOut.currentPointNum+1 <= PathModeOut.validPathNum && ... 该航段的下一航段有效
    | %         PathModeOut.currentPointNum-1 >= 1 % 前一航段有效
    | %     flag = true;
    | % end
    | 
    | %
    | %
    | % figure;
    | % % plot(minPoint1(2),minPoint1(1),'b*');hold on;
    | % % plot(minPoint2(2),minPoint2(1),'k*');hold on;
    | % plot(prepreLLA(2),prepreLLA(1),'ro');hold on;
    | % plot(preLLA(2),preLLA(1),'ro');hold on;
    | % plot(curLLA(2),curLLA(1),'ro');hold on;
    | % plot(nextLLA(2),nextLLA(1),'ro');hold on;
    | % grid on;
    | % axis equal
    | %
    | %
    | % plot(startLLA(2),startLLA(1),'r+');hold on;
    | % plot(targetLLA(2),targetLLA(1),'g+');hold on;
  function flag = isAddTransitPoint:
    | function flag = isAddTransitPoint
    | flag = false;
    | thisIdx = PathModeOut.currentPointNum;
    | if thisIdx < PathModeOut.validPathNum
    |     nextIdx = thisIdx + 1;
    | else
    |     nextIdx = thisIdx;
    | end
    | if isArrive1stPointInPathMode && ... 表示是否已经进入航线（已经到达第一个点）
    |         IN_MAV.mavlink_mission_item_def(thisIdx).param1 == 0 && IN_MAV.mavlink_mission_item_def(nextIdx).param1 ~= 0 && ... 该航段为非任务航段 且 下一航段为拍照航段（不拍照）
    |         PathModeOut.currentPointNum+1 <= PathModeOut.validPathNum && ... 该航段的下一航段有效
    |         PathModeOut.currentPointNum-1 >= 1 % 前一航段有效
    |     flag = true;
    | end
  function flag = isCompleteLoopPath:
    | function flag = isCompleteLoopPath
    | persistent numLoop
    | if isempty(numLoop)
    |     numLoop = 0;
    | end
    | numLoop = numLoop + 1;
    | printDebugInfo('PathFollow','Complete Loop Num');
    | RTInfo.Task = ENUM_RTInfo_Task.LoopPath_Complete_Num; % 更新RT信息
    | updateLogDataBuffer(ENUM_TaskLogBlockName.TASKLOG_FlightMode,RTInfo.Task,'write',[numLoop;TaskParam.loopPathPoints;0;0;0]); % 更新log缓存
    | flag = false;
    | if numLoop >= max(1,TaskParam.loopPathPoints)
    |     flag = true;
    | end
  function resetPath:
    | function resetPath
    | PathModeOut.prePointNum = PathModeOut.currentPointNum;
    | PathModeOut.currentPointNum = 2;
  function en_func:
    | function en_func
    | % Debug
    | DebugParam.stepNaviPath = 1;
    | %
    | PathModeOut.uavMode = TaskParam.uavMode_InPathFollowMode;
    | PathModeOut.flightTaskMode = ENUM_FlightTaskMode.PathFollowMode;
    | PathModeOut.flightControlMode = ENUM_FlightControlMode.PathFollowControlMode;
    | % 目标速度
    | PathModeOut.groundspeedCmd = TaskParam.cruiseSpeed_cruise;
    | % 最大爬升率
    | PathModeOut.maxClimbSpeed = TaskParam.maxClimbSpeed_fixMode;
    | PathModeOut.rollCmd = 0;
    | % 需计算指令： 
    | if isContinuePath % 继续航线模式
    |     RTInfo.Task = ENUM_RTInfo_Task.If_AutoMode_PathFollow_Init_AutoProfile_Yes; % 更新RT信息
    |     updateLogDataBuffer(ENUM_TaskLogBlockName.TASKLOG_FlightMode,RTInfo.Task,'write'); % 更新log缓存
    |     if PathModeOut.prePointNum == 0 && PathModeOut.currentPointNum == 0 % 如未初始化过，则从头走航路
    |         PathModeOut.prePointNum = idxStartPathPoint-1;
    |         PathModeOut.currentPointNum = idxStartPathPoint;
    |     else
    |         % 使用退出前的当前航路点、前置航路点信息
    |     end
    | else % 开始航线模式
    |     PathModeOut.prePointNum = idxStartPathPoint-1;
    |     PathModeOut.currentPointNum = idxStartPathPoint;
    | end
    | if PathModeOut.validPathNum == 1
    |     RTInfo.Task = ENUM_RTInfo_Task.If_AutoMode_PathFollow_Init_ValidPathNum_1; % 更新RT信息
    |     updateLogDataBuffer(ENUM_TaskLogBlockName.TASKLOG_FlightMode,RTInfo.Task,'write'); % 更新log缓存
    |     send(event_finishPath,FLIGHTMODE.AUTO_TASK.MODE_PATH);
    | elseif PathModeOut.validPathNum == 2
    |     RTInfo.Task = ENUM_RTInfo_Task.If_AutoMode_PathFollow_Init_ValidPathNum_2; % 更新RT信息
    |     updateLogDataBuffer(ENUM_TaskLogBlockName.TASKLOG_FlightMode,RTInfo.Task,'write'); % 更新log缓存
    |     send(event_goLastPoint,FLIGHTMODE.AUTO_TASK.MODE_PATH);
    | elseif PathModeOut.validPathNum > 2
    |     if PathModeOut.validPathNum ~= PathModeOut.currentPointNum
    |         if PathModeOut.currentPointNum == PathModeOut.currentPointNum % 考虑继续航点的情况
    |             RTInfo.Task = ENUM_RTInfo_Task.If_AutoMode_PathFollow_Init_ValidPathNum_n_go1st; % 更新RT信息
    |             updateLogDataBuffer(ENUM_TaskLogBlockName.TASKLOG_FlightMode,RTInfo.Task,'write'); % 更新log缓存
    |             send(event_goFirstPoint,FLIGHTMODE.AUTO_TASK.MODE_PATH);
    |         else
    |             RTInfo.Task = ENUM_RTInfo_Task.If_AutoMode_PathFollow_Init_ValidPathNum_n_goMid; % 更新RT信息
    |             updateLogDataBuffer(ENUM_TaskLogBlockName.TASKLOG_FlightMode,RTInfo.Task,'write'); % 更新log缓存
    |             send(event_goMidPoint,FLIGHTMODE.AUTO_TASK.MODE_PATH);
    |         end
    |     else
    |         send(event_goLastPoint,FLIGHTMODE.AUTO_TASK.MODE_PATH);
    |     end
    | else
    |     RTInfo.Task = ENUM_RTInfo_Task.NotDefined_State_ValidPathNum; % 更新RT信息
    |     updateLogDataBuffer(ENUM_TaskLogBlockName.TASKLOG_FlightMode,RTInfo.Task,'write'); % 更新log缓存
    |     % TODO
    | end
  function du_func:
    | function du_func
    | persistent pArriveFlag hasGenerateTurnPoint pTurnLLA distFlag
    | R = 40;
    | if isempty(pArriveFlag) || isempty(hasGenerateTurnPoint) || resetPathProgram
    |     resetPathProgram = false;
    |     pArriveFlag = -1;
    |     hasGenerateTurnPoint = false;
    |     pTurnLLA = startLLA;
    |     relpos = lla2ned(targetLLA,ComFlightOut.curLLA(1:2));
    |     dist = norm(relpos(1:2));
    |     distFlag = dist > 2*R;
    | end
    | 
    | %% ----------------- 进行路径规划
    | nextTempIdx = PathModeOut.currentPointNum + 1;
    | isWorkPoint = nextTempIdx<PathModeOut.validPathNum; %
    | smoothEnable = true; % AlgoParams.isInterpPathPoints;
    | if smoothEnable && distFlag && isWorkPoint && ...
    |         (PathModeOut.currentPointNum == 2 || (PathModeOut.currentPointNum>2 && IN_MAV.mavlink_mission_item_def(PathModeOut.currentPointNum).param1 == 0 ))
    |     nextTargetLLA = double([IN_MAV.mavlink_mission_item_def(nextTempIdx).x,...
    |         IN_MAV.mavlink_mission_item_def(nextTempIdx).y, IN_MAV.mavlink_mission_item_def(nextTempIdx).z]);
    |     tempIdx = PathModeOut.currentPointNum;
    |     targetLLA = double([IN_MAV.mavlink_mission_item_def(tempIdx).x,...
    |         IN_MAV.mavlink_mission_item_def(tempIdx).y, IN_MAV.mavlink_mission_item_def(tempIdx).z]);
    |     arriveFlag_internal = 0;
    |     if ~hasGenerateTurnPoint
    |         [turnPos,pTurnLLA,turnPointFlag] = calPreTurnPointLL(targetLLA(1:2),nextTargetLLA(1:2),startLLA(1:2),R);
    |         if ~turnPointFlag
    |             pTurnLLA = targetLLA;
    |         end
    |         hasGenerateTurnPoint = true;
    |     end
    |     if pArriveFlag == -1
    |         % 航段终点
    |         tempIdx = PathModeOut.currentPointNum;
    |         targetLLA = reshape(pTurnLLA,[1,3]);
    |         PathModeOut.prePathPoint_LLA = startLLA;
    |         PathModeOut.curPathPoint_LLA = targetLLA;
    |         % 更新PathMode输出结构体
    |         this_mission_item_def = IN_MAV.mavlink_mission_item_def(tempIdx);
    |         PathModeOut  = updatePathModeStruct(ComFlightOut.curLLA,...
    |             startLLA,  targetLLA,  PathModeOut,  this_mission_item_def);
    |         PathModeOut.dz = 0;
    |         % 判断是否到达
    |         temp_AlgoParams = TaskParam;
    |         % temp_AlgoParams.reachDetermineMode = 0; % 点判定
    |         arriveFlag_internal = double(calIfReachPoint_horizontal(ComFlightOut.curLLA,  ...
    |             startLLA,  targetLLA,  temp_AlgoParams));
    |         if arriveFlag_internal == 0
    |             arriveFlag_internal = -1;
    |         else
    |             arriveFlag_internal = 0;
    |             startLLA = ComFlightOut.curLLA;
    |         end
    |     elseif pArriveFlag == 0
    |         % 航段终点
    |         tempIdx = PathModeOut.currentPointNum;
    |         targetLLA = double([IN_MAV.mavlink_mission_item_def(tempIdx).x,...
    |             IN_MAV.mavlink_mission_item_def(tempIdx).y, IN_MAV.mavlink_mission_item_def(tempIdx).z]);
    |         PathModeOut.prePathPoint_LLA = startLLA;
    |         PathModeOut.curPathPoint_LLA = targetLLA;
    |         % 更新PathMode输出结构体
    |         this_mission_item_def = IN_MAV.mavlink_mission_item_def(tempIdx);
    |         PathModeOut  = updatePathModeStruct(ComFlightOut.curLLA,...
    |             startLLA,  targetLLA,  PathModeOut,  this_mission_item_def);
    |         PathModeOut.dz = 0;
    |         % 判断是否到达
    |         temp_AlgoParams = TaskParam;
    |         % temp_AlgoParams.reachDetermineMode = 0; % 点判定
    |         arriveFlag_internal = double(calIfReachPoint_horizontal(ComFlightOut.curLLA,  ...
    |             startLLA,  targetLLA,  temp_AlgoParams));
    |         %         if arriveFlag_internal == 0
    |         %             arriveFlag_internal = -1;
    |         %         else
    |         %             arriveFlag_internal = 0;
    |         %         end
    |     end
    | else
    |     %% ---------------- 不航路规划
    |     % 航段终点
    |     if PathModeOut.currentPointNum > 2 && IN_MAV.mavlink_mission_item_def(PathModeOut.currentPointNum).param1 ~= 0
    |         tempIdx = PathModeOut.currentPointNum-1;
    |         startLLA = double([IN_MAV.mavlink_mission_item_def(tempIdx).x,...
    |             IN_MAV.mavlink_mission_item_def(tempIdx).y, IN_MAV.mavlink_mission_item_def(tempIdx).z]);  
    |     else
    |         % 会造成起始点持续更新
    | %         startLLA = double([ComFlightOut.curLLA(1:2),mission_item_def(tempIdx).z]);
    |     end
    |     tempIdx = PathModeOut.currentPointNum;
    |     targetLLA = double([IN_MAV.mavlink_mission_item_def(tempIdx).x,...
    |         IN_MAV.mavlink_mission_item_def(tempIdx).y, IN_MAV.mavlink_mission_item_def(tempIdx).z]);
    |     PathModeOut.prePathPoint_LLA = startLLA;
    |     PathModeOut.curPathPoint_LLA = targetLLA;
    |     % 更新PathMode输出结构体
    |     this_mission_item_def = IN_MAV.mavlink_mission_item_def(tempIdx);
    |     PathModeOut  = updatePathModeStruct(ComFlightOut.curLLA,...
    |         startLLA,  targetLLA,  PathModeOut,  this_mission_item_def);
    |     if PathModeOut.currentPointNum > 2 && IN_MAV.mavlink_mission_item_def(PathModeOut.currentPointNum).param1 == 0
    |         % 若不是第一个航线点（第二个点），且不是作业点，则不控侧偏
    |         PathModeOut.dz = 0;
    |     end
    |     % 判断是否到达
    |     temp_AlgoParams = TaskParam;
    |     % temp_AlgoParams.reachDetermineMode = 0; % 点判定
    |     arriveFlag_internal = double(calIfReachPoint_horizontal(ComFlightOut.curLLA,  ...
    |         startLLA,  targetLLA,  temp_AlgoParams));
    | end
    | tempIdx = PathModeOut.currentPointNum;
    | targetLLA = double([IN_MAV.mavlink_mission_item_def(tempIdx).x,...
    |     IN_MAV.mavlink_mission_item_def(tempIdx).y, IN_MAV.mavlink_mission_item_def(tempIdx).z]);
    | distToTarget = distOfTwoLL(targetLLA(1:2),ComFlightOut.curLLA(1:2));
    | if PathModeOut.currentPointNum == 2
    |     if distToTarget < TaskParam.horiDist_verticalMove + 100
    |         PathModeOut.heightCmd = double(IN_MAV.mavlink_mission_item_def(tempIdx).z);
    |     else
    |         PathModeOut.heightCmd = double(IN_MAV.mavlink_mission_item_def(1).z);
    |     end
    | end
    | heightPoint2 = double(IN_MAV.mavlink_mission_item_def(2).z);
    | pArriveFlag = arriveFlag_internal;
    | if pArriveFlag == 1 && abs(heightPoint2-ComFlightOut.curLLA(3)) < TaskParam.vertDist_verticalMove
    |     pArriveFlag = -1;
    |     PathModeOut.prePointNum = PathModeOut.prePointNum+1;
    |     PathModeOut.currentPointNum = PathModeOut.currentPointNum+1;
    |     RTInfo.Task = ENUM_RTInfo_Task.If_AutoMode_PathFollow_Init_AutoProfile_Yes; % 更新RT信息
    |     if isDebugInfoToShow
    |         fprintf('\t\t\t time %.2f [sec]: arrive the %.0fth path point!\n',clock_sec,tempIdx);
    |     end
    |     send(event_arrivePoint,FLIGHTMODE.AUTO_TASK.MODE_PATH);
    | end
  function du_func_verticalMove:
    | function du_func_verticalMove()
    | % 判断是否需要跳转到垂直运动模式
    | tempIdx = PathModeOut.currentPointNum;
    | targetLLA = double([IN_MAV.mavlink_mission_item_def(tempIdx).x,...
    |     IN_MAV.mavlink_mission_item_def(tempIdx).y, IN_MAV.mavlink_mission_item_def(tempIdx).z]);
    | distToTarget = distOfTwoLL(targetLLA(1:2),ComFlightOut.curLLA(1:2));
    | distValue = TaskParam.horiDist_verticalMove;
    | if distToTarget < distValue && abs(PathModeOut.heightCmd - ComFlightOut.curLLA(3)) > TaskParam.vertDist_verticalMove + 5
    | %     printDebugInfo('VerticalMove Before Path','Enter Yes')
    | %     RTInfo.Task = ENUM_RTInfo_Task.VerticalMove_BeforePath_Enter_Yes; % 更新RT信息
    | %     updateLogDataBuffer(ENUM_TaskLogBlockName.TASKLOG_FlightMode,RTInfo.Task,'write',[distToTarget,distValue,ComFlightOut.curLLA(3),targetLLA(3),0]'); % 更新log缓存        
    |     send(event_verticalMove,FLIGHTMODE.AUTO_TASK);
    | else
    | %     printDebugInfo('VerticalMove Before Path','Enter No')
    | %     RTInfo.Task = ENUM_RTInfo_Task.VerticalMove_BeforePath_Enter_No; % 更新RT信息
    | %     updateLogDataBuffer(ENUM_TaskLogBlockName.TASKLOG_FlightMode,RTInfo.Task,'write',[distToTarget,distValue,ComFlightOut.curLLA(3),targetLLA(3),0]'); % 更新log缓存    
    | end
  function SendEvent_BeginPayLoadWork:
    | function SendEvent_BeginPayLoadWork
    | send(payload_beginWork,Payload)
  function SendEvent_StopPayLoadWork:
    | function SendEvent_StopPayLoadWork
    | send(payload_stopWork,Payload)
  function du_func_verticalMove:
    | function du_func_verticalMove()
    | % 判断是否需要跳转到垂直运动模式
    | tempIdx = PathModeOut.currentPointNum;
    | targetLLA = double([ComFlightOut.curHomeLLA(1),ComFlightOut.curHomeLLA(2),...
    |     IN_MAV.mavlink_mission_item_def(tempIdx).z]);
    | distToTarget = distOfTwoLL(targetLLA(1:2),ComFlightOut.curLLA(1:2));
    | if preTaskMode == ENUM_FlightTaskMode.HoverDownMode
    |     distValue = 500;
    | else
    |     distValue = TaskParam.horiDist_verticalMove;
    | end
    | if distToTarget > distValue && ...
    |         abs(targetLLA(3) - ComFlightOut.curLLA(3)) > TaskParam.vertDist_verticalMove + 10 && ...
    |         isUavInFix
    |     printDebugInfo('VerticalMove Before GoHome','Enter Yes')
    |     RTInfo.Task = ENUM_RTInfo_Task.VerticalMove_BeforeGoHome_Enter_Yes; % 更新RT信息
    |     updateLogDataBuffer(ENUM_TaskLogBlockName.TASKLOG_FlightMode,RTInfo.Task,'write',[distToTarget,distValue,ComFlightOut.curLLA(3),targetLLA(3),0]'); % 更新log缓存
    |     send(event_verticalMove,FLIGHTMODE.AUTO_TASK);
    | else
    |     printDebugInfo('VerticalMove Before GoHome','Enter No')
    |     RTInfo.Task = ENUM_RTInfo_Task.VerticalMove_BeforeGoHome_Enter_No; % 更新RT信息
    |     updateLogDataBuffer(ENUM_TaskLogBlockName.TASKLOG_FlightMode,RTInfo.Task,'write',[distToTarget,distValue,ComFlightOut.curLLA(3),targetLLA(3),0]'); % 更新log缓存
    | end
  function en_func:
    | function en_func
    | % uavMode继承前置模式
    | PathModeOut.flightTaskMode = ENUM_FlightTaskMode.GoHomeMode;
    | PathModeOut.flightControlMode = ENUM_FlightControlMode.PathFollowControlMode;
    | PathModeOut.prePointNum = PathModeOut.currentPointNum;
    | PathModeOut.currentPointNum = 1;
    | % 最大爬升率
    | if isUavInFix
    |     RTInfo.Task = ENUM_RTInfo_Task.GoHome_Approach_UavFix; % 更新RT信息
    |     updateLogDataBuffer(ENUM_TaskLogBlockName.TASKLOG_FlightMode,RTInfo.Task,'write'); % 更新log缓存
    |     PathModeOut.maxClimbSpeed = TaskParam.maxClimbSpeed_fixMode;
    | else
    |     RTInfo.Task = ENUM_RTInfo_Task.GoHome_Approach_UavRotor; % 更新RT信息
    |     updateLogDataBuffer(ENUM_TaskLogBlockName.TASKLOG_FlightMode,RTInfo.Task,'write'); % 更新log缓存
    |     PathModeOut.maxClimbSpeed = TaskParam.maxClimbSpeed_normal_TakeOffandLand;
    | end
    | % 航点信息
    | startLLA = ComFlightOut.curLLA;
    | tempIdx = 1;
    | targetLLA = double([IN_MAV.mavlink_mission_item_def(tempIdx).x,...
    |     IN_MAV.mavlink_mission_item_def(tempIdx).y, IN_MAV.mavlink_mission_item_def(tempIdx).z]);
    | distFromStartToEnd = distOfTwoLL(targetLLA(1:2),startLLA(1:2));
    | % 高度指令
    | % if distFromStartToEnd > AlgoParams.horiDist_verticalMove % 距离较远时，上升到home高度
    | %     PathModeOut.heightCmd = double(targetLLA(3));
    | % else
    |     % 捕获当前高度
    |     PathModeOut.heightCmd = double(ComFlightOut.curLLA(3));
    | %     if isUavInFix && 
    | %         
    | %     end
    | % end
  function du_func:
    | function du_func
    | % 悬停位置
    | PathModeOut.turnCenterLL = ComFlightOut.curHomeLLA(1:2);
    | tempIdx = 1; % home点序号是1
    | targetLLA = double([IN_MAV.mavlink_mission_item_def(tempIdx).x,...
    |     IN_MAV.mavlink_mission_item_def(tempIdx).y, IN_MAV.mavlink_mission_item_def(tempIdx).z]);
    | arriveFlag_tooNear = false; % 固定翼模式下如果离home点过近则不进行入行点插入
    | if isUavInFix % 
    |     if TaskParam.isHoverUpDownWithHome
    |         distFromStartToEnd = distOfTwoLL(targetLLA(1:2),startLLA(1:2));
    |         if distFromStartToEnd > 2*TaskParam.turnR
    |             % 在home点前插入一个切入点
    |             newTargetLL = calEnterLLToFlyAround(targetLLA(1:2),startLLA(1:2),TaskParam.turnR);
    |             targetLLA = [newTargetLL,targetLLA(3)];
    |         elseif distFromStartToEnd < TaskParam.turnR
    |             arriveFlag_tooNear = true;
    |         end
    |     end
    | else
    |     targetLLA = ComFlightOut.curHomeLLA;
    | end
    | % 
    | PathModeOut.prePathPoint_LLA = startLLA;
    | PathModeOut.curPathPoint_LLA = targetLLA;
    | % 航向指向home
    | PathModeOut.headingCmd = calHeadingCmd(...
    |     ComFlightOut.curLLA,  targetLLA);
    | % 设置侧偏距为0
    | PathModeOut.dz = 0;
    | % 设置预置滚转
    | PathModeOut.rollCmd = 0;
    | % 计算剩余距离
    | PathModeOut.distToGo = calPointDist_horizontal(...
    |     ComFlightOut.curLLA, targetLLA);
    | % 判断是否到达
    | temp_AlgoParams = TaskParam;
    | temp_AlgoParams.reachDetermineMode = 0; % 点判定
    | if isUavInRotor
    |     temp_AlgoParams.reachFlag_point_dist = 4;
    |     PathModeOut.groundspeedCmd = TaskParam.cruiseSpeed_rotorMode;
    | else
    |     temp_AlgoParams.reachFlag_point_dist = 15; % 进近判定
    |     PathModeOut.groundspeedCmd = TaskParam.cruiseSpeed_cruise;
    |     if PathModeOut.distToGo < 150
    |         temp_AlgoParams.reachDetermineMode = 2; % 综合判定
    |     end
    | end
    | % arriveFlag = calIfReachPoint_horizontal(ComFlightOut.curLLA,  ...
    | %     ComFlightOut.curLLA,  targetLLA,  temp_AlgoParams);
    | arriveFlag = calIfReachPoint_horizontal(ComFlightOut.curLLA,  ...
    |     startLLA,  targetLLA,  temp_AlgoParams);
    | if arriveFlag || arriveFlag_tooNear
    |     RTInfo.Task = ENUM_RTInfo_Task.If_AutoMode_GoHome_Init_Arrive; % 更新RT信息
    |     var = double([arriveFlag,arriveFlag_tooNear,0,0,0]');
    |     updateLogDataBuffer(ENUM_TaskLogBlockName.TASKLOG_FlightMode,RTInfo.Task,'write',var); % 更新log缓存
    |     if isDebugInfoToShow   
    |         fprintf('\t\t\t time %.2f [sec]: get near the home!\n',clock_sec);
    |     end
    |     send(event_getNearHome,FLIGHTMODE.AUTO_TASK.MODE_GOHOME);
    | end
  function du_func:
    | function du_func
    | switch PathModeOut.typeAutoMode
    |     case ENUM_AutoModeType.SuspendTaskToHomeThenLand
    |         RTInfo.Task = ENUM_RTInfo_Task.Switch_AutoMode_HoverAdjust_Doing_SuspendTaskToHomeThenLand; % 更新RT信息
    |         updateLogDataBuffer(ENUM_TaskLogBlockName.TASKLOG_FlightMode,RTInfo.Task,'write'); % 更新log缓存
    |         if isUavInFix
    |             printDebugInfo('GoHome','Switch SuspendTaskToHomeThenLand isUavFix')
    |             SendEvent_autoGoToNextMode
    |         else
    |             printDebugInfo('GoHome','Switch SuspendTaskToHomeThenLand isUavRotor')
    |             send(event_directToHoverFromGoHome,FLIGHTMODE.AUTO_TASK);
    |         end
    |     case ENUM_AutoModeType.SuspendTaskToHome
    |         RTInfo.Task = ENUM_RTInfo_Task.Switch_AutoMode_HoverAdjust_Doing_SuspendTaskToHome; % 更新RT信息
    |         updateLogDataBuffer(ENUM_TaskLogBlockName.TASKLOG_FlightMode,RTInfo.Task,'write'); % 更新log缓存
    |         if isUavInFix
    |             printDebugInfo('GoHome','Switch SuspendTaskToHome isUavFix')
    |             SendEvent_autoGoToNextMode
    |         else
    |             printDebugInfo('GoHome','Switch SuspendTaskToHome isUavRotor')
    |             send(event_directToHoverFromGoHome,FLIGHTMODE.AUTO_TASK);
    |         end
    |     case ENUM_AutoModeType.AutoProfile
    |         if isUavInFix
    |             printDebugInfo('GoHome','Switch AutoProfile')
    |             RTInfo.Task = ENUM_RTInfo_Task.If_AutoMode_GoHome_ToGo_AutoProfile_Yes; % 更新RT信息
    |             updateLogDataBuffer(ENUM_TaskLogBlockName.TASKLOG_FlightMode,RTInfo.Task,'write'); % 更新log缓存
    |             SendEvent_autoGoToNextMode
    |         else
    |             printDebugInfo('GoHome','Switch Otherwise isUavRotor')
    |             RTInfo.Task = ENUM_RTInfo_Task.If_AutoMode_GoHome_ToGo_AutoProfile_Yes; % 更新RT信息
    |             updateLogDataBuffer(ENUM_TaskLogBlockName.TASKLOG_FlightMode,RTInfo.Task,'write'); % 更新log缓存
    |             send(event_directToHoverFromGoHome,FLIGHTMODE.AUTO_TASK);
    |         end
    |     otherwise
    |         if isUavInFix
    |             printDebugInfo('GoHome','Switch Otherwise isUavFix')
    |             RTInfo.Task = ENUM_RTInfo_Task.If_AutoMode_GoHome_ToGo_AutoProfile_No_Fix; % 更新RT信息
    |             updateLogDataBuffer(ENUM_TaskLogBlockName.TASKLOG_FlightMode,RTInfo.Task,'write'); % 更新log缓存
    |             send(manual_airStandBy,FLIGHTMODE.AUTO_TASK);
    |         else
    |             printDebugInfo('GoHome','Switch Otherwise isUavRotor')
    |             RTInfo.Task = ENUM_RTInfo_Task.If_AutoMode_GoHome_ToGo_AutoProfile_No_Rotor; % 更新RT信息
    |             updateLogDataBuffer(ENUM_TaskLogBlockName.TASKLOG_FlightMode,RTInfo.Task,'write'); % 更新log缓存
    |             send(event_directToHoverFromGoHome,FLIGHTMODE.AUTO_TASK);
    |         end
    | end
  function ResponseEvent_manualSwitchHeight:
    | function ResponseEvent_manualSwitchHeight
    | PathModeOut.heightCmd = double(CmdParam_altitude);
    | RTInfo.Task = ENUM_RTInfo_Task.SetValue_HeightCmd; % 更新RT信息
  function setCmdWhileEnterHoverAdjustFromAirStandBy:
    | function setCmdWhileEnterHoverAdjustFromAirStandBy
    | % 保存前置模式的部分指令
    | HeightCmdBeforeAirStandBy = PathModeOut.heightCmd;
    | TaskModeBeforeAirStandBy = preTaskMode;
    | % 捕获当前高度
    | PathModeOut.heightCmd = double(ComFlightOut.curLLA(3));
    | % 
    | headingMode = 1;
    | nextMode = ENUM_FlightTaskMode.Rotor2Fix_Mode ;
  function flag = isReadyToGo:
    | function flag = isReadyToGo
    | % TODO
    | flag = 1;
    | if flag == 1
    |     if isDebugInfoToShow
    |         fprintf('\t\t\t time %.2f [sec]: HoverDown Begins!\n',clock_sec);
    |     end
    | end
  function flag = hasReachHeight:
    | function flag = hasReachHeight
    | flag = 0;
    | heightErr = ComFlightOut.curLLA(3)-PathModeOut.heightCmd;
    | if heightErr < 10
    |     flag = 1;
    |     RTInfo.Task = ENUM_RTInfo_Task.If_AutoMode_HoverDown_ReachHeight_Yes; % 更新RT信息
    |     if isDebugInfoToShow
    |         fprintf('\t\t\t time %.2f [sec]: Reach The Expected Hover Height %.0f [m]!\n',clock_sec,PathModeOut.heightCmd);
    |     end
    | end
  function flag = willSailAgainstWind:
    | function flag = willSailAgainstWind
    | persistent gsBuffer heading0_deg oneCircleComplete idxsel
    | nanflag = -9999;
    | if isempty(gsBuffer)
    |     fprintf('Start find wind\n');
    |     RTInfo_FindWind_Begin();
    |     gsBuffer = nanflag*ones(30,1);
    |     heading0_deg = ComFlightOut.curEuler(1)*180/pi;
    |     oneCircleComplete = false;
    |     idxsel = -1;
    | end
    | flag = false;
    | stepAngle = 360/length(gsBuffer);
    | curHeading_deg = ComFlightOut.curEuler(1)*180/pi;
    | vel = ComFlightOut.curWindSpeed; % ComFlightOut.curAirSpeed - ComFlightOut.curGroundSpeed;
    | diffHeading_deg = angdiff(curHeading_deg*pi/180,heading0_deg*pi/180)*180/pi;
    | if diffHeading_deg < 0
    |     diffHeading_deg = diffHeading_deg + 360;
    | end
    | 
    | if oneCircleComplete
    |     if false && all(abs(gsBuffer)<TaskParam.windSpeed_sailAgainstWindWhenBeyone)
    |         flag = true;
    |         RTInfo.FindWind = ENUM_FindWind.FW_Sail_WindIsLowerThanThreshold;
    |         fprintf('Find Wind: max windspeed < %.1f m/s\n',TaskParam.windSpeed_sailAgainstWindWhenBeyone);
    |         fprintf('Find Wind: heading %.2fdeg windspeed %.2f\n',curHeading_deg,vel);
    |     else
    |     end
    |     if abs(angdiff((idxsel-1/2)*stepAngle*pi/180,curHeading_deg*pi/180)) <= stepAngle*pi/180 && ...
    |             abs(angdiff((idxsel+1/2)*stepAngle*pi/180,curHeading_deg*pi/180)) <= stepAngle*pi/180
    |         flag = true;
    |         UpdateRTInfo_FindWind(curHeading_deg);
    |         fprintf('Find Wind: heading %.2fdeg windspeed %.2f\n',curHeading_deg,vel);
    |     end
    |     WindParamOut.sailWindSpeed = vel;
    |     WindParamOut.sailWindHeading = curHeading_deg*pi/180;
    |     WindParamOut.windSpeedMax = max(gsBuffer);
    |     WindParamOut.windSpeedMin = min(gsBuffer);
    |     WindParamOut.maxWindHeading = (idxsel-1/2)*stepAngle*pi/180;
    | end
    | 
    | for idx = 1:length(gsBuffer)
    |     %     if diffHeading_deg >= (idx-1)*stepAngle && diffHeading_deg < idx*stepAngle
    |     if curHeading_deg < 0
    |         curHeading_deg = curHeading_deg + 360;
    |     end
    |     if curHeading_deg >= (idx-1)*stepAngle && curHeading_deg < idx*stepAngle
    |         gsBuffer(idx) = vel;
    |         %         fprintf('Find Wind: [%.0f,%.0f)deg %.2f\n',(idx-1)*stepAngle,idx*stepAngle,vel)
    |     end
    | end
    | % 当收集完360度风速后，按需选择风向出航
    | if all(gsBuffer~=nanflag) && ~oneCircleComplete
    |     gsBuffer = movmean(gsBuffer,3);
    |     oneCircleComplete = true;
    |     switch TaskParam.SailModeByWind
    |         case ENUM_SailMode.AgainstWind
    |             [~,idxsel_temp] = max(gsBuffer);
    |             fprintf('One circle complete, AgainstWind\n');
    |         case ENUM_SailMode.FollowWind
    |             [~,idxsel_temp] = min(gsBuffer);
    |             fprintf('One circle complete, FollowWind\n');
    |         case ENUM_SailMode.CrossWind
    |             [~,idxsel_temp] = min(abs(gsBuffer));
    |             fprintf('One circle complete, CrossWind\n');
    |         otherwise
    |             [~,idxsel_temp] = max(gsBuffer);
    |             fprintf('One circle complete, AnyWind\n');
    |     end
    |     idxsel = idxsel_temp(1); % 防止碰巧有多个极值的情况
    |     UpdateRTInfo_SelWindSpeed(gsBuffer(idxsel));
    | end
    | % 当参数设为任意风向出航时，直接flag=ture
    | if TaskParam.SailModeByWind == ENUM_SailMode.AnyWind
    |     flag = true;
    |     RTInfo.FindWind = ENUM_FindWind.FW_OneCircleOver_AnyWind;
    | end
    | %% 子函数
    | function RTInfo_FindWind_Begin()
    | switch TaskParam.SailModeByWind
    |     case ENUM_SailMode.AgainstWind
    |         RTInfo.FindWind = ENUM_FindWind.FW_BeginFindWind_Against;
    |     case ENUM_SailMode.FollowWind
    |         RTInfo.FindWind = ENUM_FindWind.FW_BeginFindWind_Follow;
    |     case ENUM_SailMode.CrossWind
    |         RTInfo.FindWind = ENUM_FindWind.FW_BeginFindWind_Cross;
    |     otherwise
    |         RTInfo.FindWind = ENUM_FindWind.FW_BeginFindWind_Any;
    | end
    | %
    | function UpdateRTInfo_FindWind(curHeading_deg)
    | stepAngle = 30;
    | idx = 0;
    | curHeading_deg = rem(curHeading_deg,360);
    | if curHeading_deg < 0
    |     curHeading_deg = curHeading_deg + 360;
    | end
    | %
    | idx = 1;
    | if curHeading_deg > (idx-1)*stepAngle && curHeading_deg <= (idx)*stepAngle
    |     RTInfo.FindWind = ENUM_FindWind.FW_Sail_0_30_deg;
    | end
    | %
    | idx = 2;
    | if curHeading_deg > (idx-1)*stepAngle && curHeading_deg <= (idx)*stepAngle
    |     RTInfo.FindWind = ENUM_FindWind.FW_Sail_30_60_deg;
    | end
    | %
    | idx = 3;
    | if curHeading_deg > (idx-1)*stepAngle && curHeading_deg <= (idx)*stepAngle
    |     RTInfo.FindWind = ENUM_FindWind.FW_Sail_60_90_deg;
    | end
    | %
    | idx = 4;
    | if curHeading_deg > (idx-1)*stepAngle && curHeading_deg <= (idx)*stepAngle
    |     RTInfo.FindWind = ENUM_FindWind.FW_Sail_90_120_deg;
    | end
    | %
    | idx = 5;
    | if curHeading_deg > (idx-1)*stepAngle && curHeading_deg <= (idx)*stepAngle
    |     RTInfo.FindWind = ENUM_FindWind.FW_Sail_120_150_deg;
    | end
    | %
    | idx = 6;
    | if curHeading_deg > (idx-1)*stepAngle && curHeading_deg <= (idx)*stepAngle
    |     RTInfo.FindWind = ENUM_FindWind.FW_Sail_150_180_deg;
    | end
    | %
    | idx = 7;
    | if curHeading_deg > (idx-1)*stepAngle && curHeading_deg <= (idx)*stepAngle
    |     RTInfo.FindWind = ENUM_FindWind.FW_Sail_180_210_deg;
    | end
    | %
    | idx = 8;
    | if curHeading_deg > (idx-1)*stepAngle && curHeading_deg <= (idx)*stepAngle
    |     RTInfo.FindWind = ENUM_FindWind.FW_Sail_210_240_deg;
    | end
    | %
    | idx = 9;
    | if curHeading_deg > (idx-1)*stepAngle && curHeading_deg <= (idx)*stepAngle
    |     RTInfo.FindWind = ENUM_FindWind.FW_Sail_240_270_deg;
    | end
    | %
    | idx = 10;
    | if curHeading_deg > (idx-1)*stepAngle && curHeading_deg <= (idx)*stepAngle
    |     RTInfo.FindWind = ENUM_FindWind.FW_Sail_270_300_deg;
    | end
    | %
    | idx = 11;
    | if curHeading_deg > (idx-1)*stepAngle && curHeading_deg <= (idx)*stepAngle
    |     RTInfo.FindWind = ENUM_FindWind.FW_Sail_300_330_deg;
    | end
    | %
    | idx = 12;
    | if curHeading_deg > (idx-1)*stepAngle && curHeading_deg <= (idx)*stepAngle
    |     RTInfo.FindWind = ENUM_FindWind.FW_Sail_330_360_deg;
    | end
    | % 
    | function UpdateRTInfo_SelWindSpeed(windspeed)
    | if windspeed > 0 && windspeed <= 3
    |     RTInfo.FindWind = ENUM_FindWind.FW_WindSpeed_p_0_3_ms;
    | end
    | if windspeed > 3 && windspeed <= 6
    |     RTInfo.FindWind = ENUM_FindWind.FW_WindSpeed_p_3_6_ms;
    | end
    | if windspeed > 6 && windspeed <= 1e5
    |     RTInfo.FindWind = ENUM_FindWind.FW_WindSpeed_p_6_Inf_ms;
    | end
    | if windspeed > -3 && windspeed <= 0
    |     RTInfo.FindWind = ENUM_FindWind.FW_WindSpeed_m_0_3_ms;
    | end
    | if windspeed > -6 && windspeed <= -3
    |     RTInfo.FindWind = ENUM_FindWind.FW_WindSpeed_m_3_6_ms;
    | end
    | if windspeed > -1e5 && windspeed <= -6
    |     RTInfo.FindWind = ENUM_FindWind.FW_WindSpeed_m_6_Inf_ms;
    | end
  function updateDownMode:
    | function updateDownMode
    | if ~PathModeOut.isHomeChangedAfterTakeOff && ... % home点起飞后未变动
    |         ComFlightOut.curLLA(3) > 300
    |     PathModeOut.flightControlMode = ENUM_FlightControlMode.HoverSliderMode;
    | else
    |     PathModeOut.flightControlMode = ENUM_FlightControlMode.CircleHoverMode;
    | end
  function en_func_HoverDown:
    | function en_func_HoverDown
    | RTInfo.Task = ENUM_RTInfo_Task.Enter_AutoMode_HoverDown_Init; % 更新RT信息
    | updateLogDataBuffer(ENUM_TaskLogBlockName.TASKLOG_FlightMode,RTInfo.Task,'write'); % 更新log缓存
    | PathModeOut.uavMode = TaskParam.uavMode_InHoverUpDownMode;
    | updateDownMode();
    | PathModeOut.flightControlMode = ENUM_FlightControlMode.CircleHoverMode;
    | % 需计算指令： 高度 速度 滚转角 转弯半径
    | tempIdx = idxStartPathPoint;
    | if isPathDataValid && PathModeOut.typeAutoMode == ENUM_AutoModeType.AutoProfile
    |     RTInfo.Task = ENUM_RTInfo_Task.If_AutoMode_PathFollow_Init_AutoProfile_Yes; % 更新RT信息
    |     updateLogDataBuffer(ENUM_TaskLogBlockName.TASKLOG_FlightMode,RTInfo.Task,'write'); % 更新log缓存
    |     % 自动任务模式下
    |     PathModeOut.groundspeedCmd = TaskParam.cruiseSpeed_cruise;
    | else % 手动选择该模式
    |     % 捕获当前速度,设定最小值
    |     PathModeOut.groundspeedCmd = max(TaskParam.cruiseSpeed_cruise,ComFlightOut.curGroundSpeed);
    | end
    | PathModeOut.heightCmd = CmdParam_altitude;
    | % PathModeOut.turnRadiusCmd = AlgoParams.turnR;
    | PathModeOut.rollCmd = ...
    |     atan(PathModeOut.groundspeedCmd^2/PathModeOut.turnRadiusCmd/9.8);
    | % 设置侧偏距为0
    | PathModeOut.dz = 0;
    | % % 绕飞中心
    | % [dLat,dLon] = calDLatLonOfRotateCenterFromCurPos;
    | % PathModeOut.turnCenterLL =  ComFlightOut.curLLA(1:2)' + [dLat;dLon];
    | % 绕飞中心
    | if preTaskMode ~= ENUM_FlightTaskMode.HoverUpMode && ...
    |         preTaskMode ~= ENUM_FlightTaskMode.HoverDownMode
    |     if ~TaskParam.isHoverUpDownWithHome
    |         [dLat,dLon] = calDLatLonOfRotateCenterFromCurPos(...
    |             ComFlightOut.curLLA(1:2)',ComFlightOut.curEuler(1),PathModeOut.turnRadiusCmd,'right');
    |         PathModeOut.turnCenterLL =  ComFlightOut.curLLA(1:2) + [dLat,dLon];
    |     else
    |         PathModeOut.turnCenterLL =  ComFlightOut.curHomeLLA(1:2);
    |     end
    | else
    |     % 沿用HoverUpDown模式的，确保盘旋中心一致
    | end
    | % 最大爬升率
    | PathModeOut.maxClimbSpeed = TaskParam.maxClimbSpeed_fixMode;
  function du_func:
    | function du_func
    | switch PathModeOut.typeAutoMode
    |     case ENUM_AutoModeType.AutoProfile
    |         printDebugInfo('HoverDown','Switch AutoProfile')
    |         RTInfo.Task = ENUM_RTInfo_Task.If_AutoMode_HoverDown_ToGo_AutoProfile_Yes; % 更新RT信息
    |         updateLogDataBuffer(ENUM_TaskLogBlockName.TASKLOG_FlightMode,RTInfo.Task,'write'); % 更新log缓存
    |         SendEvent_autoGoToNextMode
    |         % case  ENUM_AutoModeType.SuspendTaskToLand
    |     case ENUM_AutoModeType.SuspendTaskToHome
    |         printDebugInfo('HoverDown','Switch SuspendTaskToHome')
    |         RTInfo.Task = ENUM_RTInfo_Task.If_AutoMode_HoverDown_ToGo_SuspendTaskToHome_Yes; % 更新RT信息
    |         updateLogDataBuffer(ENUM_TaskLogBlockName.TASKLOG_FlightMode,RTInfo.Task,'write'); % 更新log缓存
    |         SendEvent_autoGoToNextMode
    |         % case ENUM_AutoModeType.Fix2Rotor2HoverAdjust
    |     case ENUM_AutoModeType.SuspendTaskToHomeThenLand
    |         printDebugInfo('HoverDown','Switch SuspendTaskToHomeThenLand')
    |         RTInfo.Task = ENUM_RTInfo_Task.If_AutoMode_HoverDown_ToGo_SuspendTaskToHomeThenLand_Yes; % 更新RT信息
    |         updateLogDataBuffer(ENUM_TaskLogBlockName.TASKLOG_FlightMode,RTInfo.Task,'write'); % 更新log缓存
    |         SendEvent_autoGoToNextMode
    |     otherwise % case ENUM_AutoModeType.PauseInAir
    |         PathModeOut.rollCmd = ...
    |             atan(PathModeOut.groundspeedCmd^2/PathModeOut.turnRadiusCmd/9.8);
    |         % PathModeOut.turnRadiusCmd = AlgoParams.turnR;
    |         PathModeOut.dR_turn = calDradiusWhileTurn(PathModeOut.turnRadiusCmd,...
    |             ComFlightOut.curLLA(1:2)',PathModeOut.turnCenterLL);
    |         % 保持在当前模式
    | end
  function dist_horizontal = calPointDist_horizontal(point1LLA,point2LLA):
    | function dist_horizontal = calPointDist_horizontal(point1LLA,point2LLA)
    | % 计算水平距离
    | % point1LLA: 点1位置
    | % point2LLA: 点2位置
    | % dist: 距离 [m]
    | pos1 = lla2ned(point1LLA, point1LLA(1:2));
    | pos2 = lla2ned(point2LLA, point1LLA(1:2));
    | % 矢量
    | vec = pos2 - pos1;
    | % 距离
    | dist_horizontal = norm(vec(1:2));
  function en_func:
    | function en_func
    | % 需计算指令： 高度 航向 速度
    | tempIdx = idxStartPathPoint;
    | if isPathDataValid && PathModeOut.typeAutoMode == ENUM_AutoModeType.AutoProfile
    |     printDebugInfo('Fix2Rotor','AutoProfile Yes')
    |     RTInfo.Task = ENUM_RTInfo_Task.If_AutoMode_Fix2Rotor_Init_AutoProfile_Yes; % 更新RT信息
    |     updateLogDataBuffer(ENUM_TaskLogBlockName.TASKLOG_FlightMode,RTInfo.Task,'write'); % 更新log缓存
    |     % 自动任务模式下
    |     % 高度指令延续前一模式
    |     % 航向指令延续前一模式
    | else
    |     printDebugInfo('Fix2Rotor','AutoProfile No')
    |     % 手动选择该模式
    |     % 捕获当前航向
    |     PathModeOut.headingCmd = double(ComFlightOut.curEuler(1));
    |     % 捕获当前高度
    |     PathModeOut.heightCmd = double(ComFlightOut.curLLA(3));
    | end
    | PathModeOut.groundspeedCmd = 0;
    | % 设置侧偏距为0
    | PathModeOut.dz = 0;
    | % 设置预置滚转
    | PathModeOut.rollCmd = 0;
    | % 最大爬升率
    | PathModeOut.maxClimbSpeed = TaskParam.maxClimbSpeed_fixMode;
  function en_func_SingleMode:
    | function en_func_SingleMode
    | % 需计算指令： 高度 航向 速度
    | % 捕获当前航向
    | PathModeOut.headingCmd = double(ComFlightOut.curEuler(1));
    | % 捕获当前高度
    | PathModeOut.heightCmd = double(ComFlightOut.curLLA(3));
    | 
    | PathModeOut.groundspeedCmd = 0;
    | % 设置侧偏距为0
    | PathModeOut.dz = 0;
    | % 设置预置滚转
    | PathModeOut.rollCmd = 0;
    | % 最大爬升率
    | PathModeOut.maxClimbSpeed = TaskParam.maxClimbSpeed_fixMode;
  function flag = hasReachExpectSpeed:
    | function flag = hasReachExpectSpeed
    | speedErr = abs(ComFlightOut.curGroundSpeed - PathModeOut.groundspeedCmd);
    | flag = false;
    | if speedErr < 3
    |     flag = true;
    | end
  function SendEvent_GoTo_HoverAdjust:
    | function SendEvent_GoTo_HoverAdjust
    | send(auto_goto_HoverAdjustMode,FLIGHTMODE.AUTO_TASK);
  function flag = canEnterAirStandByMode:
    | function flag = canEnterAirStandByMode
    | % 若当前模式是固定翼，则进入AirStandBy，若当前模式是旋翼，则进入HoverAdjust
    | flag = false;
    | flag_TaskMode = PathModeOut.flightTaskMode == ENUM_FlightTaskMode.HoverUpMode || ...
    |     PathModeOut.flightTaskMode == ENUM_FlightTaskMode.HoverDownMode || ...
    |     PathModeOut.flightTaskMode == ENUM_FlightTaskMode.PathFollowMode || ...
    |     PathModeOut.flightTaskMode == ENUM_FlightTaskMode.LandMode || ...
    |     PathModeOut.flightTaskMode == ENUM_FlightTaskMode.GoHomeMode || ...
    |     PathModeOut.flightTaskMode == ENUM_FlightTaskMode.NoneFlightTaskMode || ...
    |     PathModeOut.flightTaskMode == ENUM_FlightTaskMode.AirStandByMode || ...
    |     PathModeOut.flightTaskMode == ENUM_FlightTaskMode.HoverAdjustMode || ...
    |     PathModeOut.flightTaskMode == ENUM_FlightTaskMode.TakeOffMode;
    | if PathModeOut.whereIsUAV == ENUM_Where.InTheAir && ...  % 在空中
    |        double(ComFlightOut.curLLA(3)) > TaskParam.maxClimbSpeed_nearGround_TakeOffandLand && ... % 当前高度大于xx m
    |        flag_TaskMode % 容许的前置任务模式
    |     flag = true; 
    | else
    |     printComInfo('canEnterAirStandByMode() False',0)
    | end
  function updateLandMaxHeight:
    | function updateLandMaxHeight
    | persistent preLandMaxHeight
    | %% 重置 -------------------------------------------------------------------
    | persistent preTakeOffNum
    | if isempty(preTakeOffNum)
    |     preTakeOffNum = PathModeOut.numTakeOff;
    | end
    | if isempty(preLandMaxHeight) || preTakeOffNum ~= PathModeOut.numTakeOff
    |     preTakeOffNum = PathModeOut.numTakeOff;
    | %% 重置END ----------------------------------------------------------------   
    |     preLandMaxHeight = ComFlightOut.curLLA(3);
    | end
    | if ComFlightOut.curLLA(3) > preLandMaxHeight
    |     preLandMaxHeight = ComFlightOut.curLLA(3);
    | end
    | RTInfo.landMaxHeight = preLandMaxHeight;
  function flag = isReadyToLand:
    | function flag = isReadyToLand
    | persistent heightRecord
    | num = 10;
    | %% 重置 -------------------------------------------------------------------
    | persistent preTakeOffNum
    | if isempty(preTakeOffNum)
    |     preTakeOffNum = PathModeOut.numTakeOff;
    | end
    | if isempty(heightRecord) || preTakeOffNum ~= PathModeOut.numTakeOff
    |     preTakeOffNum = PathModeOut.numTakeOff;
    | %% 重置END ----------------------------------------------------------------   
    |     heightRecord = zeros(1,num);
    | end
    | flag = false;
    | curHeight = ComFlightOut.curLLA(3);
    | if curHeight >= 0 && curHeight < 1
    |     heightRecord(1) = 1;
    | elseif curHeight >= 1 && curHeight < 2
    |     heightRecord(2) = 1;
    | elseif curHeight >= 2 && curHeight < 3
    |     heightRecord(3) = 1;
    | elseif curHeight >= 3 && curHeight < 4
    |     heightRecord(4) = 1;
    | elseif curHeight >= 4 && curHeight < 5
    |     heightRecord(5) = 1;
    | elseif curHeight >= 5 && curHeight < 6
    |     heightRecord(6) = 1;
    | elseif curHeight >= 6 && curHeight < 7
    |     heightRecord(7) = 1;
    | elseif curHeight >= 7 && curHeight < 8
    |     heightRecord(8) = 1;    
    | elseif curHeight >= 8 && curHeight < 9
    |     heightRecord(9) = 1;
    | elseif curHeight >= 9 && curHeight < 10
    |     heightRecord(10) = 1;        
    | end
    | if sum(heightRecord)>num-2 && heightRecord(1) == 1
    |     flag = true;
    | end
  function en_func:
    | function en_func
    | % 悬停位置
    | PathModeOut.turnCenterLL = ComFlightOut.curLLA(1:2) + moveLandMark; % 不能省略
    | % PathModeOut.turnCenterLL = ComFlightOut.curLLA(1:2); 
    | switch PathModeOut.typeAutoMode
    |     case {ENUM_AutoModeType.SuspendTaskToHomeThenLand,ENUM_AutoModeType.Fix2Rotor2Home2Land}
    |         RTInfo.Task = ENUM_RTInfo_Task.Switch_AutoMode_Land_NearGround_SuspendTaskToHomeThenLand; % 更新RT信息
    |         PathModeOut.turnCenterLL = ComFlightOut.curHomeLLA(1:2) + moveLandMark;
    |     case  ENUM_AutoModeType.SuspendTaskToLand
    |         RTInfo.Task = ENUM_RTInfo_Task.Switch_AutoMode_Land_NearGround_SuspendTaskToLand; % 更新RT信息
    |         %         if ~isAnyGPSOk
    |         %             PathModeOut.turnCenterLL = ComFlightOut.curLLA(1:2)';
    |         %         end
    |     case ENUM_AutoModeType.SuspendTaskToHome
    |         %     case {ENUM_AutoModeType.SuspendTaskToHome,ENUM_AutoModeType.SuspendTaskToHomeThenLand}
    |         RTInfo.Task = ENUM_RTInfo_Task.Switch_AutoMode_Land_NearGround_SuspendTaskToHome; % 更新RT信息
    |         PathModeOut.turnCenterLL = ComFlightOut.curHomeLLA(1:2) + moveLandMark;
    |     case ENUM_AutoModeType.AutoProfile
    |         RTInfo.Task = ENUM_RTInfo_Task.Switch_AutoMode_Land_NearGround_AutoProfile; % 更新RT信息
    |         if nextMode == ENUM_FlightTaskMode.LandMode
    |             PathModeOut.turnCenterLL = ComFlightOut.curHomeLLA(1:2) + moveLandMark;
    |         end
    |     otherwise
    |         RTInfo.Task = ENUM_RTInfo_Task.NotDefined_State_Land_NearGround_Switch; % 更新RT信息
    | end
  function [flag,dist] = hasReachLatLon_assign(posErr):
    | function [flag,dist] = hasReachLatLon_assign(posErr)
    | flag = false;
    | tempdLL = moveLandMark;
    | dLat = PathModeOut.turnCenterLL(1) + tempdLL(1)- ComFlightOut.curLLA(1);
    | dLon = PathModeOut.turnCenterLL(2) + tempdLL(2)- ComFlightOut.curLLA(2);
    | deg2m = 111e3;
    | dPn = dLat*deg2m;
    | dPe = dLon*deg2m*cos(ComFlightOut.curLLA(1)*pi/180);
    | dist = norm([dPn,dPe]);
    | if dist < posErr
    |     flag = true;
    | end
  function flag = hasLanded:
    | function flag = hasLanded
    | flag = false;
    | % cond1 = (ComFlightOut.curLLA(3) < AlgoParams.heightThreshold_LandSuccess && (isHitGround));
    | radarFlag = isRadarHeightContinue;
    | cond1 = (ComFlightOut.curLLA(3) < TaskParam.heightThreshold_LandSuccess+0.1 && IN_NAVI.hitGroundByAccZ);
    | cond2 = (ComFlightOut.curLLA(3) < 0.9*TaskParam.heightThreshold_LandSuccess && radarFlag);
    | cond3 = isNearGroundLong && radarFlag;
    | if IN_SignalIntegrity.SensorStatus.radar1 == ENUM_SensorHealthStatus.Health || ...
    |         isUm482Good(IN_SENSOR.um482.BESTPOS)
    |     % 高精度测高：radar正常或差分GPS正常
    |     if cond1 || cond2 || cond3
    |         flag = true;
    |     end
    | else
    |     % 
    | end
    | if cond1
    |     RTInfo.LandCond1_Acc_H = true;
    |     RTInfo.Task = ENUM_RTInfo_Task.Land_HasLandCond_Acc_H; % 更新RT信息
    |     updateLogDataBuffer(ENUM_TaskLogBlockName.TASKLOG_FlightMode, RTInfo.Task,'write'); % 更新log缓存
    |     fprintf('Land Completed: LandCond1_Acc_H, height %.3fm,Az %.0fm/s^2,Vd %.3f\n',ComFlightOut.curLLA(3),IN_SENSOR.IMU1.accel_z,ComFlightOut.curVelNED(3));
    | end
    | if cond2
    |     RTInfo.LandCond1_Vd_H = true;
    |     RTInfo.Task = ENUM_RTInfo_Task.Land_HasLandCond_H_Continue; % 更新RT信息
    |     updateLogDataBuffer(ENUM_TaskLogBlockName.TASKLOG_FlightMode, RTInfo.Task,'write'); % 更新log缓存
    |     fprintf('Land Completed: LandCond1_Vd_H, height %.3fm,Az %.0fm/s^2,Vd %.3f\n',ComFlightOut.curLLA(3),IN_SENSOR.IMU1.accel_z,ComFlightOut.curVelNED(3));
    | end
    | if cond3
    |     RTInfo.LandCond3_near = true;
    |     RTInfo.Task = ENUM_RTInfo_Task.Land_HasLandCond_NearGround_Continue; % 更新RT信息
    |     updateLogDataBuffer(ENUM_TaskLogBlockName.TASKLOG_FlightMode, RTInfo.Task,'write'); % 更新log缓存
    |     fprintf('Land Completed: LandCond3_near, height %.3fm,Az %.0fm/s^2,Vd %.3f\n',ComFlightOut.curLLA(3),IN_SENSOR.IMU1.accel_z,ComFlightOut.curVelNED(3));
    | end
  function flag = hasReachNearGroundHeight:
    | function flag = hasReachNearGroundHeight
    | flag = false;
    | heightErr = ComFlightOut.curLLA(3)-TaskParam.midHeight_TakeOffandLand;
    | if heightErr < 4
    |     flag = true;
    |     RTInfo.Task = ENUM_RTInfo_Task.If_AutoMode_Land_ReachHeight_Yes; % 更新RT信息
    | end
  function flag = isRadarHeightContinue:
    | function flag = isRadarHeightContinue
    | persistent heightHistory_step1 heightHistory_step2
    | %% 重置 -------------------------------------------------------------------
    | persistent preTakeOffNum
    | if isempty(preTakeOffNum)
    |     preTakeOffNum = PathModeOut.numTakeOff;
    | end
    | if isempty(heightHistory_step1) || preTakeOffNum ~= PathModeOut.numTakeOff
    |     preTakeOffNum = PathModeOut.numTakeOff;
    | %% 重置END ----------------------------------------------------------------    
    |     heightHistory_step1 = false;
    |     heightHistory_step2 = false;
    | end
    | flag = false;
    | h = ComFlightOut.curLLA(3);
    | % step1
    | h0 = TaskParam.heightThreshold_LandSuccess + 0.3;
    | h1 = TaskParam.heightThreshold_LandSuccess + 0.6;
    | if RTInfo.landMaxHeight > h0
    |     if inSpan(h,h0,h1) && ~heightHistory_step1
    |         heightHistory_step1 = true;
    |         printComInfo('Land step 1',1)
    |     end
    | else
    |     heightHistory_step1 = true;
    | end
    | % step2
    | h0 = TaskParam.heightThreshold_LandSuccess + 0.6;
    | h1 = TaskParam.heightThreshold_LandSuccess + 0.9;
    | if RTInfo.landMaxHeight > h0
    |     if inSpan(h,h0,h1) && ~heightHistory_step2
    |         heightHistory_step2 = true;
    |         printComInfo('Land step 2',1)
    |     end
    | else
    |     heightHistory_step2 = true;
    | end
    | % all
    | if heightHistory_step1 && ...
    |         heightHistory_step2
    |     flag = true;
    |     RTInfo.radarHeightContinueFlag = true;
    | %     printComInfo('Land step all',1)
    | end
    | 
    | function flag = inSpan(h,h0,h1)
    | if h >= h0 && h < h1
    |     flag = true;
    | else
    |     flag = false;
    | end
  function flag = isNearGroundLong:
    | function flag = isNearGroundLong
    | persistent duration
    | %% 重置 -------------------------------------------------------------------
    | persistent preTakeOffNum
    | if isempty(preTakeOffNum)
    |     preTakeOffNum = PathModeOut.numTakeOff;
    | end
    | if isempty(duration) || preTakeOffNum ~= PathModeOut.numTakeOff
    |     preTakeOffNum = PathModeOut.numTakeOff;
    | %% 重置END ----------------------------------------------------------------    
    |     duration = 0;
    | end
    | flag = false;
    | if abs(ComFlightOut.curLLA(3)) < 0.3 % m/s^2, 注意符号，静止时z轴加速度计值为+9.8左右
    |     duration = duration + 1;
    | else
    |     duration = 0;
    | end
    | if duration >= round(3/Ts)
    |     flag = true;
    |     printComInfo('H < 0.15m for 3sec',1)
    | end
  function du_func_eval:
    | function du_func_eval
    | persistent preDist preNum_Land
    | persistent preTakeOffNum
    | if isempty(preTakeOffNum)
    |     preTakeOffNum = PathModeOut.numTakeOff;
    | end
    | if isempty(preDist) || preTakeOffNum ~= PathModeOut.numTakeOff
    |     preTakeOffNum = PathModeOut.numTakeOff;
    |     preDist = 0;
    |     preNum_Land = enterNum_Land;
    | end
    | % 最大爬升率
    | % radarHeight = double(IN_SENSOR.radar1.Range);
    | % if IN_SignalIntegrity.SensorStatus.radar1 == ENUM_SensorHealthStatus.Health || ...
    | %         isUm482Good(IN_SENSOR.um482.BESTPOS)
    | %     PathModeOut.maxClimbSpeed = AlgoParams.maxClimbSpeed_normal_TakeOffandLand;
    | % else
    | %     PathModeOut.maxClimbSpeed = AlgoParams.maxClimbSpeed_nearGround_TakeOffandLand;
    | % end
    | tempHomeLLA = ComFlightOut.curHomeLLA(1:2) + moveLandMark;
    | switch PathModeOut.typeAutoMode
    |     case {ENUM_AutoModeType.SuspendTaskToHomeThenLand,ENUM_AutoModeType.Fix2Rotor2Home2Land}
    |         RTInfo.Task = ENUM_RTInfo_Task.Switch_AutoMode_Land_NearGround_SuspendTaskToHomeThenLand; % 更新RT信息
    |         PathModeOut.turnCenterLL = tempHomeLLA;
    |     case  ENUM_AutoModeType.SuspendTaskToLand
    |         RTInfo.Task = ENUM_RTInfo_Task.Switch_AutoMode_Land_NearGround_SuspendTaskToLand; % 更新RT信息
    |         if ~isAnyGPSOk
    |             PathModeOut.turnCenterLL = tempHomeLLA;
    |         end
    |     case ENUM_AutoModeType.SuspendTaskToHome
    |         RTInfo.Task = ENUM_RTInfo_Task.Switch_AutoMode_Land_NearGround_SuspendTaskToHome; % 更新RT信息
    |         PathModeOut.turnCenterLL = tempHomeLLA;
    |     case ENUM_AutoModeType.AutoProfile
    |         RTInfo.Task = ENUM_RTInfo_Task.Switch_AutoMode_Land_NearGround_AutoProfile; % 更新RT信息
    |         if nextMode == ENUM_FlightTaskMode.LandMode
    |             PathModeOut.turnCenterLL = tempHomeLLA;
    |         end
    |     otherwise
    |         RTInfo.Task = ENUM_RTInfo_Task.NotDefined_State_Land_NearGround_Switch; % 更新RT信息
    | end
    | distThreshold = 6;
    | [~,dist] =  hasReachLatLon_assign(distThreshold);
    | isLatLonOK_Land = false;
    | if ~TaskParam.isLandMarkMoving
    |     if (dist > distThreshold && preDist <= distThreshold) ||...
    |             (dist > distThreshold && preNum_Land ~= enterNum_Land)
    |         % 捕获当前高度
    |         send(event_goHomeThenLand_LargeOffsetInLand,FLIGHTMODE.AUTO_TASK)
    |         %     PathModeOut.heightCmd = double(ComFlightOut.curLLA(3));
    |     elseif hasReachLatLon_assign(3)
    |         PathModeOut.heightCmd = TaskParam.midHeight_TakeOffandLand;
    |         isLatLonOK_Land = true;
    |     end
    | else
    |     isLatLonOK_Land = true;
    | end
    | preDist = dist;
    | preNum_Land = enterNum_Land;
  function flag = isUm482Good(bestpos):
    | function flag = isUm482Good(bestpos)
    | if bestpos == ENUM_BESTPOS.POS_SOLUTION_PSRDIFF || ...
    |         bestpos == ENUM_BESTPOS.POS_SOLUTION_L1_INT || ...
    |         bestpos == ENUM_BESTPOS.POS_SOLUTION_WIDE_INT || ...
    |         bestpos == ENUM_BESTPOS.POS_SOLUTION_NARROW_INT || ...
    |         bestpos == ENUM_BESTPOS.POS_SOLUTION_L1_FLOATE || ...
    |         bestpos == ENUM_BESTPOS.POS_SOLUTION_NARROW_FLOATE
    |     flag = true;
    | else
    |     flag = false;
    | end
  function en_func:
    | function en_func
    | switch PathModeOut.typeAutoMode
    |     case ENUM_AutoModeType.SuspendTaskToHomeThenLand
    |         printDebugInfo('Land','Switch SuspendTaskToHomeThenLand')
    |         RTInfo.Task = ENUM_RTInfo_Task.Switch_AutoMode_Land_NearGround_SuspendTaskToHomeThenLand; % 更新RT信息
    |     case  ENUM_AutoModeType.SuspendTaskToLand
    |         printDebugInfo('Land','Switch SuspendTaskToLand')
    |         RTInfo.Task = ENUM_RTInfo_Task.Switch_AutoMode_Land_NearGround_SuspendTaskToLand; % 更新RT信息
    |     case ENUM_AutoModeType.SuspendTaskToHome
    |         printDebugInfo('Land','Switch SuspendTaskToHome')
    |         RTInfo.Task = ENUM_RTInfo_Task.Switch_AutoMode_Land_NearGround_SuspendTaskToHome; % 更新RT信息
    |     case ENUM_AutoModeType.AutoProfile
    |         printDebugInfo('Land','Switch AutoProfile')
    |         RTInfo.Task = ENUM_RTInfo_Task.Switch_AutoMode_Land_NearGround_AutoProfile; % 更新RT信息
    |     otherwise
    |         printDebugInfo('Land','Switch Otherwise')
    |         RTInfo.Task = ENUM_RTInfo_Task.NotDefined_State_Land_NearGround_Switch; % 更新RT信息
    | end
  function du_update_Center:
    | function du_update_Center
    | if TaskParam.isLandMarkMoving
    |     PathModeOut.turnCenterLL = ComFlightOut.curLLA(1:2) + moveLandMark;
    | end
  function du_update_HeightCmd:
    | function du_update_HeightCmd
    | persistent preDist preNum_Land
    | if isempty(preDist)
    |     preDist = 0;
    |     preNum_Land = enterNum_Land;
    | end
    | distThreshold = 4;
    | [~,dist] = hasReachLatLon_assign(distThreshold);
    | isLatLonOK_Land = false;
    | 
    | PathModeOut.heightCmd = TaskParam.heightCmd_FinalLand;
    | if (dist > distThreshold && preDist <= distThreshold) || (dist > distThreshold && preNum_Land ~= enterNum_Land) && ...
    |         ~isLandUncondition % 电池电量耗尽判断
    |     % 捕获当前高度
    |     PathModeOut.heightCmd = double(ComFlightOut.curLLA(3));
    | elseif hasReachLatLon_assign(2)
    |     isLatLonOK_Land = true;
    | end
    | preDist = dist;
    | preNum_Land = enterNum_Land;
  function du_update_VdCmd:
    | function du_update_VdCmd
    | persistent pVdCmd preVdCmd 
    | persistent preTakeOffNum
    | if isempty(preTakeOffNum)
    |     preTakeOffNum = PathModeOut.numTakeOff;
    | end
    | if isempty(pVdCmd) || preTakeOffNum ~= PathModeOut.numTakeOff
    |     preTakeOffNum = PathModeOut.numTakeOff;
    |     pVdCmd = TaskParam.maxClimbSpeed_nearGround_TakeOffandLand;
    |     preVdCmd = pVdCmd;
    | end
    | Kbase1 = 2/5;
    | Kbase2 = 7/25;
    | d = 3; % AlgoParams.VdCmdSwitchHeight_NearGroundWhenLand之上d[m]开始减速
    | if ComFlightOut.curLLA(3) > 15 
    |     VdCmd = TaskParam.maxClimbSpeed_normal_TakeOffandLand;
    | elseif ComFlightOut.curLLA(3) < TaskParam.VdCmdSwitchHeight_NearGroundWhenLand && ...
    |         ComFlightOut.curLLA(3) >= 3/5*TaskParam.VdCmdSwitchHeight_NearGroundWhenLand
    |     VdCmd = Kbase1*TaskParam.maxClimbSpeed_nearGround_TakeOffandLand;
    | elseif ComFlightOut.curLLA(3) < 3/5*TaskParam.VdCmdSwitchHeight_NearGroundWhenLand
    |     VdCmd = Kbase2*TaskParam.maxClimbSpeed_nearGround_TakeOffandLand;
    | else
    |     VdCmd = TaskParam.maxClimbSpeed_nearGround_TakeOffandLand;
    | end
    | kk = 0.92;
    | pVdCmd = kk*pVdCmd + (1-kk)*VdCmd;
    | if pVdCmd > preVdCmd
    |     pVdCmd = preVdCmd;
    | else
    |     preVdCmd = pVdCmd;
    | end
    | PathModeOut.maxClimbSpeed = pVdCmd;
  function out = moveLandMark:
    | function out = moveLandMark
    | persistent dLat dLon dPx dPy
    | if isempty(dLat)
    |     dLat = 0;
    |     dLon = 0;
    |     dPx = 0;
    |     dPy = 0;
    | end
    | if TaskParam.isLandMarkMoving ~= TaskParam.nanFlag
    |     kk = 1e3;
    |     R = 6378e3;
    |     curLat = ComFlightOut.curLLA(1);
    |     heading = pi/180*rem(TaskParam.isLandMarkMoving,kk);
    |     speed = double(int16(TaskParam.isLandMarkMoving/kk));
    |     maxSpeed = 10;
    |     if speed > maxSpeed
    |         speed = maxSpeed;
    |     elseif speed < -maxSpeed
    |         speed = -maxSpeed;
    |     end
    |     dPx = dPx + Ts*speed*cos(heading);
    |     dPy = dPy + Ts*speed*sin(heading);
    |     dLat = dLat + Ts*speed*cos(heading)/R*180/pi;
    |     dLon = dLon + Ts*speed*sin(heading)/R/cos(curLat*pi/180)*180/pi;
    |     pause = 1;
    | end
    | % fprintf('slassddd %.6f\t%.6f\n',dLat,dLon);
    | % fprintf('slassddd %.2f\t%.2f\n',dPx,dPy);
    | out = [dLat,dLon];
  function SendEvent_ContinueFromPause:
    | function SendEvent_ContinueFromPause
    | RTInfo.Task = ENUM_RTInfo_Task.Enter_AutoMode_Fcn_ContinueFromPause; % 更新RT信息
    | PathModeOut.flightTaskMode = TaskModeBeforeAirStandBy;
    | PathModeOut.heightCmd = HeightCmdBeforeAirStandBy;
    | PathModeOut.typeAutoMode = typeAutoModePre;
    | switch PathModeOut.flightTaskMode
    |     case ENUM_FlightTaskMode.HoverUpMode
    |         RTInfo.Task = ENUM_RTInfo_Task.Switch_AutoMode_Fcn_ContinueFromPause_HoverUp; % 更新RT信息
    |         send(manual_hoverUp,FLIGHTMODE.AUTO_TASK);
    |     case ENUM_FlightTaskMode.HoverDownMode
    |         RTInfo.Task = ENUM_RTInfo_Task.Switch_AutoMode_Fcn_ContinueFromPause_HoverDown; % 更新RT信息
    |         send(manual_hoverDown,FLIGHTMODE.AUTO_TASK);
    |     case ENUM_FlightTaskMode.PathFollowMode
    |         RTInfo.Task = ENUM_RTInfo_Task.Switch_AutoMode_Fcn_ContinueFromPause_PathFollow; % 更新RT信息
    |         send(manual_goIntoPath,FLIGHTMODE.AUTO_TASK);
    |     case ENUM_FlightTaskMode.TakeOffMode
    |         RTInfo.Task = ENUM_RTInfo_Task.Switch_AutoMode_Fcn_ContinueFromPause_TakeOff; % 更新RT信息
    |         send(manual_rotorGoUp,FLIGHTMODE.AUTO_TASK);
    |     case ENUM_FlightTaskMode.LandMode
    |         RTInfo.Task = ENUM_RTInfo_Task.Switch_AutoMode_Fcn_ContinueFromPause_Land; % 更新RT信息
    |         send(manual_land,FLIGHTMODE.AUTO_TASK);
    |     case ENUM_FlightTaskMode.GoHomeMode
    |         RTInfo.Task = ENUM_RTInfo_Task.Switch_AutoMode_Fcn_ContinueFromPause_GoHome; % 更新RT信息
    |         send(manual_goHomePoint,FLIGHTMODE.AUTO_TASK);
    |     case ENUM_FlightTaskMode.HoverAdjustMode
    |         RTInfo.Task = ENUM_RTInfo_Task.Switch_AutoMode_Fcn_ContinueFromPause_HoverAdjust; % 更新RT信息
    |         send(manual_hoverAdjust,FLIGHTMODE.AUTO_TASK);
    |     case ENUM_FlightTaskMode.NoneFlightTaskMode
    |         % do nothing
    |         RTInfo.Task = ENUM_RTInfo_Task.Switch_AutoMode_Fcn_ContinueFromPause_NoneMode; % 更新RT信息
    |     otherwise
    |         RTInfo.Task = ENUM_RTInfo_Task.NotDefined_Fcn_ContinueFromPause; % 更新RT信息
    | end
  function flag = isReadyToGo:
    | function flag = isReadyToGo
    | % TODO
    | flag = 1;
    | if flag == 1
    |     if isDebugInfoToShow
    |         fprintf('\t\t\t time %.2f [sec]: AirStandBy Begins!\n',clock_sec);
    |     end
    | end
  function flag = isHeadingToTarget:
    | function flag = isHeadingToTarget
    | flag = false;
    | errAngle = angdiff(ComFlightOut.curEuler(1),HeadingCmdBeforeAirStandBy);
    | fprintf('%.2f\n',errAngle*57.3)
    | if abs(errAngle)<20*pi/180
    |     flag = true;
    |     printDebugInfo('AirStandBy','Already Heading To Target',2)
    | end
  function en_func_AirStandBy:
    | function en_func_AirStandBy
    | % 需计算指令： 高度 速度 滚转角 转弯半径
    | tempIdx = idxStartPathPoint;
    | if PathModeOut.typeAutoMode == ENUM_AutoModeType.AutoProfile || ...
    |         PathModeOut.typeAutoMode == ENUM_AutoModeType.SuspendTaskToLand || ...
    |         PathModeOut.typeAutoMode == ENUM_AutoModeType.SuspendTaskToHome
    |     RTInfo.Task = ENUM_RTInfo_Task.If_AutoMode_AirStandBy_Init_AutoProfile_Yes; % 更新RT信息
    |     updateLogDataBuffer(ENUM_TaskLogBlockName.TASKLOG_FlightMode, RTInfo.Task,'write'); % 更新log缓存
    |     % 自动任务模式下
    |     test = 1;
    | else
    |     % 捕获当前速度,设定最小值
    |     PathModeOut.groundspeedCmd = max(TaskParam.cruiseSpeed_cruise,ComFlightOut.curGroundSpeed);
    |     % 捕获当前高度,设定最小值
    |     PathModeOut.heightCmd = max(TaskParam.minHeightInFix,double(ComFlightOut.curLLA(3)));
    | end
    | % PathModeOut.turnRadiusCmd = AlgoParams.turnR;
    | PathModeOut.rollCmd = ...
    |     atan(PathModeOut.groundspeedCmd^2/PathModeOut.turnRadiusCmd/9.8);
    | % 设置侧偏距为0
    | PathModeOut.dz = 0;
    | % 绕飞中心
    | if preTaskMode ~= ENUM_FlightTaskMode.HoverUpMode && ...
    |         preTaskMode ~= ENUM_FlightTaskMode.HoverDownMode
    |     [dLat,dLon] = calDLatLonOfRotateCenterFromCurPos(...
    |         ComFlightOut.curLLA(1:2)',ComFlightOut.curEuler(1),PathModeOut.turnRadiusCmd,'right');
    |     PathModeOut.turnCenterLL =  ComFlightOut.curLLA(1:2) + [dLat,dLon];
    | else
    |     % 沿用HoverUpDown模式的
    | end
    | % 最大爬升率
    | PathModeOut.maxClimbSpeed = TaskParam.maxClimbSpeed_fixMode;
  function flag = hasReachHeight:
    | function flag = hasReachHeight
    | flag = false;
    | heightErr = abs(ComFlightOut.curLLA(3)-PathModeOut.heightCmd);
    | if heightErr < 3
    |     flag = true;
    | %     RTInfo.Task = ENUM_RTInfo_Task.If_AutoMode_HoverAdjust_ReachHeight_Yes; % 更新RT信息
    | %     if isDebugInfoToShow
    | %         fprintf('\t\t\t time %.2f [sec]: Reach The Expected Hover Height %.0f [m]!\n',clock_sec,PathModeOut.heightCmd);
    | %     end
    | end
  function en_func:
    | function en_func
    | printDebugInfo('StallRecovery','StablizePitchAndRoll')
    | RTInfo.Task = ENUM_RTInfo_Task.Enter_AutoMode_StallRecovery_StablizePitchAndRoll; % 更新RT信息
    | updateLogDataBuffer(ENUM_TaskLogBlockName.TASKLOG_FlightMode, RTInfo.Task,'write'); % 更新log缓存
    | PathModeOut.uavMode = ENUM_UAVMode.Rotor;
    | PathModeOut.flightTaskMode = ENUM_FlightTaskMode.StallRecovery;
    | PathModeOut.flightControlMode = ENUM_FlightControlMode.OnlyStablizePitchAndRoll;
    | % 捕获当前航向
    | PathModeOut.headingCmd = double(ComFlightOut.curEuler(1));
    | % 捕获当前高度
    | PathModeOut.heightCmd = double(ComFlightOut.curLLA(3));
    | % 地速
    | PathModeOut.groundspeedCmd = 0;
    | % 设置侧偏距为0
    | PathModeOut.dz = 0;
    | % 设置预置滚转
    | PathModeOut.rollCmd = 0;
    | % 悬停位置
    | PathModeOut.turnCenterLL = ComFlightOut.curLLA(1:2);
    | % 最大爬升率
    | PathModeOut.maxClimbSpeed = TaskParam.maxClimbSpeed_normal_TakeOffandLand;
  function flag = hasReachLatLon:
    | function flag = hasReachLatLon
    | flag = false;
    | dLat = PathModeOut.turnCenterLL(1)- ComFlightOut.curLLA(1);
    | dLon = PathModeOut.turnCenterLL(2)- ComFlightOut.curLLA(2);
    | deg2m = 111e3;
    | dPn = dLat*deg2m;
    | dPe = dLon*deg2m*cos(ComFlightOut.curLLA(1)*pi/180);
    | dist = norm([dPn,dPe]);
    | if dist < 3
    |     flag = true;
    | %     RTInfo.Task = ENUM_RTInfo_Task.If_AutoMode_HoverAdjust_ReachHeight_Yes; % 更新RT信息
    | %     if isDebugInfoToShow
    | %         fprintf('\t\t\t time %.2f [sec]: Reach The Expected Hover Height %.0f [m]!\n',clock_sec,PathModeOut.heightCmd);
    | %     end
    | end
  function flag = hasMatchAllConditons:
    | function flag = hasMatchAllConditons
    | flag = false;
    | if hasReachHeight && hasReachLatLon && isAttitudeStable_globalvar
    |     flag = true;
    |     RTInfo.Task = ENUM_RTInfo_Task.If_AutoMode_HoverAdjust_ReachHeightAndLevelPoint_Yes; % 更新RT信息
    |     if isDebugInfoToShow
    |         fprintf('\t\t\t time %.2f [sec]: Reach The Expected Hover Height %.0f [m] and Level Point (%.6f, %.6f)!\n',...
    |             clock_sec,PathModeOut.heightCmd,PathModeOut.turnCenterLL(1),PathModeOut.turnCenterLL(2));
    |     end
    | end
  function flag = isPitchRollStable:
    | function flag = isPitchRollStable
    | flag = false;
    | if abs(ComFlightOut.curEuler(2)) < 15*pi/180 && ...
    |     abs(ComFlightOut.curEuler(3)) < 15*pi/180
    |     flag =true;
    | end
  function flag = isPitchRollStableLongEnough:
    | function flag = isPitchRollStableLongEnough
    | flag = false;
    | duration = clock_sec - stableTime0;
    | if duration > 1.5 % sec
    |     flag =true;
    | end
  function en_func:
    | function en_func
    | PathModeOut.heightCmd = double(IN_MAV.mavlink_mission_item_def(PathModeOut.currentPointNum).z);
    | PathModeOut.flightTaskMode = ENUM_FlightTaskMode.VerticalMove;
    | PathModeOut.flightControlMode = ENUM_FlightControlMode.CircleHoverMode;
    | switch PathModeOut.uavMode
    |     case ENUM_UAVMode.Fix
    |         PathModeOut.turnRadiusCmd = TaskParam.turnR;
    |         PathModeOut.rollCmd = ...
    |             atan(PathModeOut.groundspeedCmd^2/PathModeOut.turnRadiusCmd/9.8);
    |         % 绕飞中心
    |         [dLat,dLon] = calDLatLonOfRotateCenterFromCurPos(...
    |             ComFlightOut.curLLA(1:2)',ComFlightOut.curEuler(1),PathModeOut.turnRadiusCmd,'right');
    |         PathModeOut.turnCenterLL =  ComFlightOut.curLLA(1:2) + [dLat,dLon];
    |     otherwise
    |         PathModeOut.turnCenterLL =  ComFlightOut.curLLA(1:2);
    | end
    | 
    | % 最大爬升率
    | PathModeOut.maxClimbSpeed = TaskParam.maxClimbSpeed_fixMode;
    | 
    | % switch preTaskMode
    | %     case ENUM_FlightTaskMode.
  function du_func:
    | function du_func
    | PathModeOut.dR_turn = calDradiusWhileTurn(PathModeOut.turnRadiusCmd,...
    |     ComFlightOut.curLLA(1:2)',PathModeOut.turnCenterLL);
  function flag = reachHeight:
    | function flag = reachHeight
    | flag = false;
    | if abs(PathModeOut.heightCmd - ComFlightOut.curLLA(3)) < TaskParam.vertDist_verticalMove
    |     flag = true; 
    | end
  function flag = isHeadingToTarget:
    | function flag = isHeadingToTarget
    | flag = false;
    | switch preTaskMode
    |     case ENUM_FlightTaskMode.PathFollowMode % 退出条件：当前航向与本模式进入航行一致
    |         errAngle = angdiff(ComFlightOut.curEuler(1),headingIN_VerticalMove);
    |     case ENUM_FlightTaskMode.GoHomeMode % 退出条件：当前航向指向home点
    |         tempIdx = 1;
    |         targetLLA = double([IN_MAV.mavlink_mission_item_def(tempIdx).x,...
    |             IN_MAV.mavlink_mission_item_def(tempIdx).y, IN_MAV.mavlink_mission_item_def(tempIdx).z]);
    |         headingCmd = calHeadingCmd(ComFlightOut.curLLA,  targetLLA);
    |         errAngle = angdiff(ComFlightOut.curEuler(1),headingCmd);
    |     otherwise
    |         errAngle = angdiff(ComFlightOut.curEuler(1),headingIN_VerticalMove);
    | end
    | % errAngle = angdiff(ComFlightOut.curEuler(1),headingIN_VerticalMove);
    | if abs(errAngle) < 20*pi/180
    |     flag = true;
    |     printDebugInfo('VerticalMove','Already Heading To Target',2)
    | end
  function du_func:
    | function du_func
    | switch preTaskMode
    |     case ENUM_FlightTaskMode.PathFollowMode
    |         send(manual_goIntoPath,FLIGHTMODE.AUTO_TASK);
    |     case ENUM_FlightTaskMode.GoHomeMode
    |         send(manual_goHomePoint,FLIGHTMODE.AUTO_TASK);
    |     otherwise
    |         send(manual_goHomePoint,FLIGHTMODE.AUTO_TASK);
    | end
  function du_func_manual:
    | function du_func_manual
    | if ComFlightOut.curGroundSpeed < 10 % 只是一个粗略判断，并不真的表示在手动模式中飞机是固定翼or旋翼
    |     PathModeOut.uavMode = ENUM_UAVMode.Rotor;
    | else
    |     PathModeOut.uavMode = ENUM_UAVMode.Fix;
    | end
    | %
    | if (ComFlightOut.curLLA(3) < 5 && ComFlightOut.curGroundSpeed < 2) || ...
    |         (IN_SENSOR.radar1.Range < 1 && IN_SignalIntegrity.SensorStatus.radar1 == ENUM_SensorHealthStatus.Health)
    |     PathModeOut.whereIsUAV = ENUM_Where.OnGround;
    | else
    |     PathModeOut.whereIsUAV = ENUM_Where.InTheAir;
    | end
  function initHomeParam:
    | function initHomeParam
    | HomeParam.altitudeHome = double(IN_NAVI.lla(3));
    | HomeParam.llaHome = double(IN_NAVI.lla);
    | HomeParam.baroHeightHome = double(IN_SENSOR.baro1.alt_baro);
  function en_func:
    | function en_func
    | % HomeParam;
  function flag  = doTakePicture:
    | function flag  = doTakePicture
    | persistent picLLA
    | if isempty(picLLA)
    |     picLLA = ComFlightOut.curLLA;
    | end
    | % 位置计算
    | curPos = lla2ned(ComFlightOut.curLLA, ComFlightOut.curLLA(1:2));
    | lastPos = lla2ned(picLLA, ComFlightOut.curLLA(1:2));
    | tempIdx = PathModeOut.prePointNum;
    | prePathPointLLA = double([IN_MAV.mavlink_mission_item_def(tempIdx).x,...
    |     IN_MAV.mavlink_mission_item_def(tempIdx).y, IN_MAV.mavlink_mission_item_def(tempIdx).z]);
    | tempIdx = PathModeOut.currentPointNum;
    | curPathPointLLA = double([IN_MAV.mavlink_mission_item_def(tempIdx).x,...
    |     IN_MAV.mavlink_mission_item_def(tempIdx).y, IN_MAV.mavlink_mission_item_def(tempIdx).z]);
    | curPathPointPos = lla2ned(curPathPointLLA, ComFlightOut.curLLA(1:2));
    | prePathPointPos = lla2ned(prePathPointLLA, ComFlightOut.curLLA(1:2));
    | curPos(3) = 0;
    | lastPos(3) = 0;
    | flag = false;
    | dist = norm(curPos-lastPos);
    | % if dist > CmdParam_cameraTrigDist-Ts*ComFlightOut.curGroundSpeed && isAttitudeStable_globalvar && abs(PathModeOut.dz) < 10 && ...
    | %         abs(angdiff(PathModeOut.headingCmd,ComFlightOut.curEuler(1))) < 15*pi/180
    | lenOfThisPath = norm(curPathPointPos(1:2)-prePathPointPos(1:2));
    | distToTarget = norm(curPathPointPos(1:2)-curPos(1:2));
    | % kk = ComFlightOut.curGroundSpeed/(AlgoParams.cruiseSpeed_cruise+eps);
    | % if isnan(kk)
    | %     kk = 1;
    | % end
    | % kk = min(2,kk);
    | % kk = max(0.5,kk);
    | if dist > CmdParam_cameraTrigDist-Ts*ComFlightOut.curGroundSpeed ... % 拍照间隔条件
    |         && abs(PathModeOut.dz) < 10 % 侧偏距条件
    |     tempIdx = PathModeOut.currentPointNum;
    |     thisPathparam1 = IN_MAV.mavlink_mission_item_def(tempIdx).param1;
    |     if tempIdx > 1
    |         tempPreIdx = tempIdx - 1;
    |         prePathparam1 = double(IN_MAV.mavlink_mission_item_def(tempPreIdx).param1);
    |     else
    |         prePathparam1 = 0;
    |     end
    |     if prePathparam1 == 2
    |         flag = true;
    |         picLLA = ComFlightOut.curLLA;
    |     else
    |         if distToTarget < lenOfThisPath - TaskParam.reachFlag_point_dist % 提前结束拍照
    |             flag = true;
    |             picLLA = ComFlightOut.curLLA;
    |         end
    |     end
    | end
  function initCameraStruct:
    | function initCameraStruct
    | PayloadControlOut.CAMERA.time = 0;
    | PayloadControlOut.CAMERA.trigger = 0;
    | PayloadControlOut.CAMERA.LLA = [0;0;0];
    | PayloadControlOut.CAMERA.groundspeed = 0;
  function flag = isOnGround:
    | function flag = isOnGround
    | flag = false;
    | if PathModeOut.whereIsUAV == ENUM_Where.OnGround
    |     flag = true;
    | end
  function flag = isAttitudeStable_Alevel:
    | function flag = isAttitudeStable_Alevel
    | persistent rollset pitchset
    | if isempty(rollset)
    |     num = min(ceil(1/Ts),100); % 等效60*0.036 = 2sec
    |     rollset = -999*ones(num,1);
    |     pitchset = -999*ones(num,1);
    | end
    | flag = false;
    | rollset(2:end) = rollset(1:end-1);
    | pitchset(2:end) = pitchset(1:end-1);
    | 
    | rollset(1) = ComFlightOut.curEuler(3);
    | pitchset(1) = ComFlightOut.curEuler(2);
    | 
    | if max(abs(rollset(:))) <= 10*pi/180 && ...
    |         max(abs(pitchset(:))) <= 20*pi/180
    |     flag = true;
    | end
  function flag = isAllowedToTakeOff:
    | function flag = isAllowedToTakeOff
    | flag = true;
    | flag1 = IN_SignalIntegrity.SystemHealthStatus ~= ENUM_SystemHealthStatus.SystemHealth;
    | flag2 = PathModeOut.typeAutoMode == ENUM_AutoModeType.NotAutoMode;
    | flag3 = BatteryOut.batteryStatus ~= ENUM_BatteryStatus.BatteryNormal;
    | flag4 = isNotInFense;
    | flag5 = ~isComNormal;
    | flag6 = ~isOnGround;
    | flag7 = ~isNaviFilterStart;
    | flag8 = ~isPathDataValid;
    | flag9 = ~isUavInRotor;
    | if IN_SignalIntegrity.SystemHealthStatus ~= ENUM_SystemHealthStatus.SystemHealth || ... % 传感器不正常
    |         PathModeOut.typeAutoMode == ENUM_AutoModeType.NotAutoMode || ... % 处于非自动模式
    |         BatteryOut.batteryStatus ~= ENUM_BatteryStatus.BatteryNormal || ... % 电池电量低
    |         isNotInFense || ... % 不处于电子篱笆范围内
    |         ~isComNormal || ...% 地面站与遥控器通信断开
    |         ~isOnGround || ... % 飞机不在地面
    |         ~isNaviFilterStart || ... % 组合导航滤波器初始化完成
    |         ~isPathDataValid || ... 
    |         ~isUavInRotor % 飞机不是旋翼模式            
    |     flag = false;
    | end
    | num = 2^1*flag1 + ...
    |       2^2*flag2 + ...
    |       2^3*flag3 + ...
    |       2^4*flag4 + ...
    |       2^5*flag5 + ...
    |       2^6*flag6 + ...
    |       2^7*flag7 + ...
    |       2^8*flag8 + ...
    |       2^9*flag9;
    | if num > 0
    |     RTInfo.Task = ENUM_RTInfo_Task.Not_Allowed_TakeOff; % 更新RT信息
    |     updateLogDataBuffer(ENUM_TaskLogBlockName.TASKLOG_FlightMode,RTInfo.Task,'write',[num;0;0;0;0;]); % 更新log缓存
    | end
  function flag = isPathDataValid:
    | function flag = isPathDataValid
    | % 判断航线数据是否有效
    | persistent numPathPoints
    | if isempty(numPathPoints)
    |     numPathPoints = PathModeOut.validPathNum;
    | end
    | if numPathPoints ~= PathModeOut.validPathNum
    |     printComInfo('Path Changes',0)
    | end
    | flag = false;
    | if PathModeOut.validPathNum > 1
    |     flag = true;
    | else
    |     %     printComInfo('Path Point Num is %.0f, Not Allowed',0,PathModeOut.validPathNum)
    | end
    | numPathPoints = PathModeOut.validPathNum;
    | for i = 1:TaskParam.maxPathPointNum - 1
    |     if i <= PathModeOut.validPathNum
    |         if IN_MAV.mavlink_mission_item_def(i).x == IN_MAV.mavlink_mission_item_def(i+1).x && ... % 当连续两个航点的经纬度相等时
    |                 IN_MAV.mavlink_mission_item_def(i).y == IN_MAV.mavlink_mission_item_def(i+1).y
    |             if 0 % 暂时屏蔽
    |                 flag = false;
    |             end
    |             %             fprintf('Invalid PathPoints, %.0fth Points == the next Point\n',i);
    |             printComInfo('Invalid PathPoints, %.0fth Points == the next Point',i)
    |             %             send(event_oneKeyGoHome,FLIGHTMODE.AUTO_TASK)
    |         end
    |     else
    |         break
    |     end
    | end
  function p = lla2ned(lla, ll0):
    | function p = lla2ned(lla, ll0)
    | % 纬经高转换为NED位置
    | % lla: 纬度[deg] 经度[deg] 高度[m] 
    | % ll0: 基准点， 纬度[deg] 经度[deg]
    | % p: NED位置
    | p = zeros(1,3);
    | psi0 = 0;
    | href = 0;
    | f = 0.003352810664747;
    | R = 6378.137e3;
    | % wrap latitude and longitude if needed
    | [~, lla(:,1), lla(:,2)] = wraplatitude( lla(:,1), lla(:,2), 'deg' );
    | [~, ll0(1), ll0(2)] = wraplatitude( ll0(1), ll0(2), 'deg' );
    | 
    | % check and fix angle wrapping in longitude
    | [~, lla(:,2)] = wraplongitude( lla(:,2), 'deg', '180' );
    | [~, ll0(2)] = wraplongitude( ll0(2), 'deg', '180' );
    | 
    | dLat = lla(:,1) - ll0(1);
    | dLon = lla(:,2) - ll0(2);
    | 
    | % wrap latitude and longitude if needed
    | [~, dLat, dLon] = wraplatitude( dLat', dLon', 'deg' );
    | 
    | % check and fix angle wrapping in longitude
    | [~, dLon] = wraplongitude( dLon, 'deg', '180' );
    | 
    | rll0 = ll0*pi/180;
    | rpsi0 = psi0*pi/180;
    | 
    | Rn = R/sqrt(1-(2*f-f*f)*sin(rll0(1))*sin(rll0(1)));
    | Rm = Rn*((1-(2*f-f*f))/(1-(2*f-f*f)*sin(rll0(1))*sin(rll0(1))));
    | 
    | dNorth = dLat./atan2(1,Rm)*pi/180;
    | dEast = dLon./atan2(1,Rn*cos(rll0(1)))*pi/180;
    | 
    | p(:,1) = cos(rpsi0)*dNorth + sin(rpsi0)*dEast;
    | p(:,2) = -sin(rpsi0)*dNorth + cos(rpsi0)*dEast;
    | p(:,3) = -lla(:,3) - href;
    | end
    | 
    | function [lat_wrapped, lat, lon] = wraplatitude( lat, lon, units)
    | % WRAPLATITUDE internal function to check and fix angle wrapping in
    | % latitude and longitude if needed.
    | 
    | %   Copyright 2007-2013 The MathWorks, Inc.
    | 
    | % Convert units if necessary
    | if strcmp(units,'deg')
    |     pideg = 180;
    | else
    |     pideg = pi;
    | end
    | 
    | % Set lat_wrapped flag to false
    | lat_wrapped = false;
    | 
    | % Re-set latitudes to values between pi and -pi
    | flat = abs(lat);
    | 
    | if any(flat>pideg)
    |     lat(flat>pideg) = mod(lat(flat>pideg)+pideg,2*pideg)-pideg;
    |     % Set lat_wrapped flag to true if necessary
    |     flat = abs(lat);
    |     lat_wrapped = true;
    | end
    | 
    | % Determine if any latitudes need to be wrapped
    | idx = flat>pideg/2;
    | 
    | if any(idx)
    |     
    |     % Adjustments for -pi to pi
    |     flat = abs(lat);
    |     latp2 = flat>pideg/2;
    |     lon(idx) = lon(idx) + pideg;
    |     lat(latp2) = sign(lat(latp2)).*(pideg/2-(flat(latp2)-pideg/2));
    |     
    |     % Set lat_wrapped flag to true if necessary
    |     lat_wrapped = true;
    |     
    | end
    | end
    | 
    | function [lon_wrapped, lon] = wraplongitude( lon, inputUnits, maxRange )
    | % WRAPLONGITUDE internal function to check and fix angle wrapping in
    | % longitude.
    | 
    | %   Copyright 2007-2010 The MathWorks, Inc.
    | 
    | % Convert units if necessary
    | if strcmp(inputUnits,'deg')
    |     lon = lon*pi/180;
    | end
    | 
    | lon_wrapped = false;
    | 
    | switch maxRange
    |     % Range goes between -pi and pi
    |     case {'180','pi'}
    |         idx = lon > pi | lon < -pi;
    |         if any(idx)
    |             lon(idx) = rem(lon(idx),2*pi)- (2*pi)*fix(rem(lon(idx),2*pi)/pi);
    |             lon_wrapped = true;
    |         end
    |     % Range goes between 0 and 2*pi
    |     case {'360','2*pi'}
    |         idx = lon > 2*pi | lon < 0;
    |         if any(idx)
    |             lon(idx) = mod(lon(idx),2*pi);
    |             lon_wrapped = true;
    |         end
    |     otherwise
    |         % do nothing
    | end
    | 
    | % Convert units if necessary
    | if strcmp(inputUnits,'deg')
    |     lon = lon*180/pi;
    | end
    | end
  function flag = isOutOfFense(fenseDist):
    | function flag = isOutOfFense(fenseDist)
    | flag = false;
    | relativePosFromHome = lla2ned(ComFlightOut.curLLA, ComFlightOut.curHomeLLA(1:2));
    | relativePosFromHome(3) = 0;
    | distFromHome = norm(relativePosFromHome);
    | if distFromHome >= fenseDist% 大于5km
    |     flag = true;
    | %     LLA = ComFlightOut.curLLA;
    | end
  function initInputCmdParam:
    | function initInputCmdParam
    | % 逻辑控制参数初始化，若需通过cmd修改，则应增加相应的mavlink指令
    | isContinuePath = false;
    | idxStartPathPoint = 2; % 默认以第idxStartPoint个航点为起始航点
    | % 与高度切换命令共同作用，高度切换后，高度指令在当前任务模式下将不受的任务预设值影响
    | doHeightCmdKeepAfterHeightSwitch = false; 
    | CmdParam_cameraTrigDist = 20;
    | CmdParam_altitude = TaskParam.finalHeight_TakeOff;
    | hasTaskStarted_globalbar = false;
    | isNotInFense = false;
    | isComNormal = true;
    | landPosMode = ENUM_LandMode.HomeVTL;
    | hasTakeOff = false;
  function flag = isHomeChangeAfterTakeOff:
    | function flag = isHomeChangeAfterTakeOff
    | % 判断航线数据是否有效
    | persistent preHome pFlag
    | if isempty(preHome)
    |     preHome = [IN_MAV.mavlink_mission_item_def(1).x,IN_MAV.mavlink_mission_item_def(1).y,IN_MAV.mavlink_mission_item_def(1).z];
    |     pFlag = false;
    | end
    | newHome = [IN_MAV.mavlink_mission_item_def(1).x,IN_MAV.mavlink_mission_item_def(1).y,IN_MAV.mavlink_mission_item_def(1).z];
    | relPos = lla2ned(preHome, newHome(1:2));
    | dist = norm(relPos(1:2));
    | if dist > 50 && hasTakeOff
    |     pFlag = true;
    | end
    | flag = pFlag;
  function initBatteryOut:
    | function initBatteryOut
    | BatteryOut.mileage = 0;
    | BatteryOut.remainingMileage = 0;
    | BatteryOut.remainingTimeSec = 0;
  function increaseMileage:
    | function increaseMileage
    | % 计算飞行里程
    | persistent preLLA
    | if isempty(preLLA)
    |     preLLA = ComFlightOut.curLLA;
    | end
    | curPos = lla2ned(ComFlightOut.curLLA, ComFlightOut.curLLA(1:2));
    | lastPos = lla2ned(preLLA, ComFlightOut.curLLA(1:2));
    | curPos(3) = 0;
    | lastPos(3) = 0;
    | if isMoving
    |     dMileage = norm(curPos-lastPos);
    |     preLLA = ComFlightOut.curLLA;
    |     BatteryOut.mileage = BatteryOut.mileage + dMileage;
    | end
  function flag  = isMoving:
    | function flag  = isMoving
    | flag = false;
    | if ComFlightOut.curGroundSpeed > 1
    |     flag = true; 
    | end
  function flag = hasReadValidOnPlaneStoreData:
    | function flag = hasReadValidOnPlaneStoreData
    | flag = false;
    | if IN_ONPLANESTORE.isDataValid
    |     flag = true;
    | end
  function initAllData:
    | function initAllData
    | OUT_ONPLANESTORE.mileage_m = 0;
    | % 
    | OUT_ONPLANESTORE.Number.sortie = uint16(0);
    | OUT_ONPLANESTORE.Number.nTakeOff = uint16(0);
    | OUT_ONPLANESTORE.Number.nPowerOn = uint16(1);
    | OUT_ONPLANESTORE.Number.nPath = uint16(0);
    | OUT_ONPLANESTORE.Number.nLand = uint16(0);
    | OUT_ONPLANESTORE.Number.nRotor2Fix = uint16(0);
    | OUT_ONPLANESTORE.Number.nFix2Rotor = uint16(0);
    | 
    | OUT_ONPLANESTORE.Duration.fixInAir = 0;
    | OUT_ONPLANESTORE.Duration.rotorInAir = 0;
    | OUT_ONPLANESTORE.Duration.rotorOnGround = 0;
    | OUT_ONPLANESTORE.Duration.fixAirSpeed_0_10 = 0;
    | OUT_ONPLANESTORE.Duration.fixAirSpeed_10_20 = 0;
    | OUT_ONPLANESTORE.Duration.fixAirSpeed_20_30 = 0;
    | OUT_ONPLANESTORE.Duration.fixAirSpeed_30_40 = 0;
    | OUT_ONPLANESTORE.Duration.rotorSpeed_0_5 = 0;
    | OUT_ONPLANESTORE.Duration.rotorSpeed_5_10 = 0;
    | OUT_ONPLANESTORE.Duration.rotorSpeed_10_20 = 0;
    | OUT_ONPLANESTORE.Duration.rotorSpeed_20_30 = 0;
  function updataData:
    | function updataData
    | OUT_ONPLANESTORE.mileage_m = BatteryOut.mileage;
    | switch PathModeOut.uavMode
    |     case ENUM_UAVMode.Fix
    |         if PathModeOut.whereIsUAV == ENUM_Where.InTheAir
    |             OUT_ONPLANESTORE.Duration.fixInAir = OUT_ONPLANESTORE.Duration.fixInAir + Ts;
    |             tempSpeed = ComFlightOut.curAirSpeed;
    |             if tempSpeed <= 10
    |                 OUT_ONPLANESTORE.Duration.fixAirSpeed_0_10 = OUT_ONPLANESTORE.Duration.fixAirSpeed_0_10 + Ts;
    |             elseif tempSpeed > 10 && tempSpeed <= 20
    |                 OUT_ONPLANESTORE.Duration.fixAirSpeed_10_20 = OUT_ONPLANESTORE.Duration.fixAirSpeed_10_20 + Ts;
    |             elseif tempSpeed > 20 && tempSpeed <= 30
    |                 OUT_ONPLANESTORE.Duration.fixAirSpeed_20_30 = OUT_ONPLANESTORE.Duration.fixAirSpeed_20_30 + Ts;
    |             elseif tempSpeed > 30 && tempSpeed <= 40
    |                 OUT_ONPLANESTORE.Duration.fixAirSpeed_30_40 = OUT_ONPLANESTORE.Duration.fixAirSpeed_30_40 + Ts;
    |             end
    |         end
    |     case ENUM_UAVMode.Rotor
    |         if PathModeOut.whereIsUAV == ENUM_Where.InTheAir
    |             OUT_ONPLANESTORE.Duration.rotorInAir = OUT_ONPLANESTORE.Duration.rotorInAir + Ts;
    |             tempSpeed = ComFlightOut.curGroundSpeed;
    |             if tempSpeed <= 5
    |                 OUT_ONPLANESTORE.Duration.rotorSpeed_0_5 = OUT_ONPLANESTORE.Duration.rotorSpeed_0_5 + Ts;
    |             elseif tempSpeed > 5 && tempSpeed <= 10
    |                 OUT_ONPLANESTORE.Duration.rotorSpeed_5_10 = OUT_ONPLANESTORE.Duration.rotorSpeed_5_10 + Ts;
    |             elseif tempSpeed > 10 && tempSpeed <= 20
    |                 OUT_ONPLANESTORE.Duration.rotorSpeed_10_20 = OUT_ONPLANESTORE.Duration.rotorSpeed_10_20 + Ts;
    |             elseif tempSpeed > 20 && tempSpeed <= 30
    |                 OUT_ONPLANESTORE.Duration.rotorSpeed_20_30 = OUT_ONPLANESTORE.Duration.rotorSpeed_20_30 + Ts;
    |             end
    |         else
    |             OUT_ONPLANESTORE.Duration.rotorOnGround = OUT_ONPLANESTORE.Duration.rotorOnGround + Ts;
    |         end
    | end
    | 
    | % on exit(FLIGHTMODE.AUTO_TASK.MODE_TAKEOFF):
    | %     OUT_ONPLANESTORE.Number.sortie = OUT_ONPLANESTORE.Number.sortie + 1;
    | %     OUT_ONPLANESTORE.Number.nTakeOff = OUT_ONPLANESTORE.Number.nTakeOff + 1;
    | % on exit(FLIGHTMODE.AUTO_TASK.MODE_PATH):
    | %     OUT_ONPLANESTORE.Number.nPath = OUT_ONPLANESTORE.Number.nPath + 1;
    | % on exit(FLIGHTMODE.AUTO_TASK.MODE_LAND):
    | %     OUT_ONPLANESTORE.Number.nLand = OUT_ONPLANESTORE.Number.nLand + 1;
    | % on exit(FLIGHTMODE.AUTO_TASK.MODE_ROTOR2FIX):
    | %     OUT_ONPLANESTORE.Number.nRotor2Fix = OUT_ONPLANESTORE.Number.nRotor2Fix + 1;
    | % on exit(FLIGHTMODE.AUTO_TASK.MODE_FIX2ROTOR):
    | %     OUT_ONPLANESTORE.Number.nFix2Rotor = OUT_ONPLANESTORE.Number.nFix2Rotor + 1;
  function out = m2lat(pos):
    | function out = m2lat(pos)
    | k = 111e3;
    | out = 1/k*pos;
  function printComInfo(debugInfo,tabspace,varargin):
    | function printComInfo(debugInfo,tabspace,varargin)
    | if nargin == 3
    |     value = double(varargin{1});
    |     noValue = false;
    | else
    |     value = 0;
    |     noValue = true;
    | end
    | if isDebugInfoToShow
    |     if ~noValue
    |         switch tabspace
    |             case 0
    |                 fprintf([' %.3f sec: ',debugInfo,'\n'],clock_sec,value);
    |             case 1
    |                 fprintf(['\t %.3f sec: ',debugInfo,'\n'],clock_sec,value);
    |             case 2
    |                 fprintf(['\t\t %.3f sec: ',debugInfo,'\n'],clock_sec,value);
    |             case 3
    |                 fprintf(['\t\t\t %.3f sec: ',debugInfo,'\n'],clock_sec,value);
    |             case 4
    |                 fprintf(['\t\t\t\t %.3f sec: ',debugInfo,'\n'],clock_sec,value);
    |         end
    |     else
    |         switch tabspace
    |             case 0
    |                 fprintf([' %.3f sec: ',debugInfo,'\n'],clock_sec);
    |             case 1
    |                 fprintf(['\t %.3f sec: ',debugInfo,'\n'],clock_sec);
    |             case 2
    |                 fprintf(['\t\t %.3f sec: ',debugInfo,'\n'],clock_sec);
    |             case 3
    |                 fprintf(['\t\t\t %.3f sec: ',debugInfo,'\n'],clock_sec);
    |             case 4
    |                 fprintf(['\t\t\t\t %.3f sec: ',debugInfo,'\n'],clock_sec);
    |         end        
    |     end
    | end
  function out = m2lon(pos,lat_deg):
    | function out = m2lon(pos,lat_deg)
    | k = 111e3;
    | lat_rad = lat_deg*pi/180;
    | out = 1/k/cos(lat_rad)*pos;
  function printDebugInfo(modeName,debugInfo,varargin):
    | function printDebugInfo(modeName,debugInfo,varargin)
    | if nargin == 3
    |     tabspace = varargin{1};
    | else
    |     tabspace = 2;
    | end
    | if isDebugInfoToShow
    |     switch tabspace
    |         case 0
    |             fprintf(' %.3f sec: [%s] %s\n',clock_sec,modeName,debugInfo);
    |         case 1
    |             fprintf('\t %.3f sec: [%s] %s\n',clock_sec,modeName,debugInfo);
    |         case 2
    |             fprintf('\t\t %.3f sec: [%s] %s\n',clock_sec,modeName,debugInfo);
    |         case 3
    |             fprintf('\t\t\t %.3f sec: [%s] %s\n',clock_sec,modeName,debugInfo);
    |         case 4
    |             fprintf('\t\t\t\t %.3f sec: [%s] %s\n',clock_sec,modeName,debugInfo);
    |     end
    | end
  function flag = isNaviFilterStart:
    | function flag = isNaviFilterStart
    | flag = false;
    | % 
    | headingRotateFlag = PathModeOut.isHeadingRotate_OnGround;
    | % if IN_NAVI.initialAlignmentCompleteFlag && IN_NAVI.isNavFilterGood && ~headingRotateFlag
    | if IN_NAVI.initialAlignmentCompleteFlag && ~headingRotateFlag
    |     flag = true;
    | end
    | RTInfo.NaviStatus = ENUM_NaviStatus.NaviNormal; % 更新RT信息
    | if ~IN_NAVI.initialAlignmentCompleteFlag
    |     RTInfo.NaviStatus = ENUM_NaviStatus.NaviNotInitial; % 更新RT信息
    | else
    |     if headingRotateFlag
    |         RTInfo.NaviStatus = ENUM_NaviStatus.NaviBad_OnGround; % 更新RT信息
    |     end
    | end
  function initPathModeOut:
    | function initPathModeOut
    | persistent initFlag
    | if isempty(initFlag)
    |     initFlag = 0;
    | end
    | % 初始化stateflow内部结构体
    | PathModeOut.currentPointNum = 0;
    | PathModeOut.prePointNum = 0;
    | % PathModeOut.validPathNum = 0;
    | PathModeOut.headingCmd = 0;
    | PathModeOut.distToGo = 0;
    | PathModeOut.dz = 0;
    | PathModeOut.groundspeedCmd = 0;
    | PathModeOut.rollCmd = 0;
    | PathModeOut.turnRadiusCmd = TaskParam.turnR;   
    | PathModeOut.heightCmd = 0;
    | PathModeOut.turnCenterLL = [0,0];
    | PathModeOut.dR_turn = 0;
    | % PathModeOut.uavMode = ENUM_UAVMode.NoneUAVMode;
    | % PathModeOut.flightTaskMode = ENUM_FlightTaskMode.NoneFlightTaskMode;
    | % PathModeOut.flightControlMode = ENUM_FlightControlMode.NoneFlightControlMode;
    | % PathModeOut.AutoManualMode = ENUM_ControlMode.Auto;
    | PathModeOut.whereIsUAV = ENUM_Where.OnGround;
    | PathModeOut.typeAutoMode = ENUM_AutoModeType.NotAutoMode; 
    | PathModeOut.LLATaskInterrupt = [0;0;0];
    | PathModeOut.isTaskComplete = false;
    | PathModeOut.numTakeOff = 0;
    | PathModeOut.isAllowedToPause = true;
    | PathModeOut.isAirspeedGood = true;
    | PathModeOut.airspeedOffset = TaskParam.airspeedOffset;
    | preTaskMode = ENUM_FlightTaskMode.GroundStandByMode;
  function flag = isAllBatteryLow:
    | function flag = isAllBatteryLow
    | flag = false;
    | %% 条件1：电池电量低于阈值
    | nBattery = length(IN_MAV.mavlink_msg_mission_current);
    | for i = 1:nBattery
    |     if IN_MAV.mavlink_msg_mission_current(i).remaining <= TaskParam.low_battery_alarm_set
    |         % 如果任意一个电池电量低于预设值
    |         flag = true;
    |         break
    |     end
    | end
    | %% 条件2：收到飞行性能模块发送的需返航标志
    | if isNeedToGoHomeNow && TaskParam.enableDynamicBatteryGoHome
    |     flag = true;
    | end
  function flag = isAllBatterySevereLow:
    | function flag = isAllBatterySevereLow
    | flag = false;
    | nBattery = length(IN_MAV.mavlink_msg_mission_current);
    | for i = 1:nBattery
    |     if IN_MAV.mavlink_msg_mission_current(i).remaining <= TaskParam.severe_low_battery_alarm_set
    |         % 如果任意一个电池电量低于预设值
    |         flag = true;
    |         break
    |     end
    | end
  function flag = isNeedToGoHomeNow:
    | function flag = isNeedToGoHomeNow
    | % 仅在固定翼下的正常航线模式或暂停模式下触发
    | flag = false;
    | if IN_FlightPerf.flagGoHomeNow % && isUavInFix && ...
    | %         (PathModeOut.typeAutoMode == ENUM_AutoModeType.AutoProfile || PathModeOut.typeAutoMode == ENUM_AutoModeType.PauseInAir)
    |     % 如果任意一个电池电量低于预设值
    |     flag = true;
    | end
  function flag = enforceLand:
    | function flag = enforceLand
    | persistent idx
    | if isempty(idx)
    |     idx = 0;
    | end
    | % 当电量低至耗尽阈值时，若此时非降落模式，则触发一次降落事件
    | flag = false;
    | nBattery = length(IN_MAV.mavlink_msg_mission_current);
    | if idx == 0 % 只运行一次
    |     if PathModeOut.flightTaskMode ~= ENUM_FlightTaskMode.LandMode
    |         for i = 1:nBattery
    |             % 当电量低至耗尽阈值时
    |             if IN_MAV.mavlink_msg_mission_current(i).remaining == TaskParam.runout_battery_alarm_set
    |                 flag = true;
    |                 idx = idx + 1;
    |                 break
    |             end
    |         end
    |     end
    |     if flag
    |         curBattery = double(IN_MAV.mavlink_msg_mission_current(1).remaining);
    |         threshBattery = double(TaskParam.runout_battery_alarm_set);
    |         RTInfo.Task = ENUM_RTInfo_Task.TaskLog_Protect_Battery_RunOut;% 更新RTInfo Task
    |         updateLogDataBuffer(ENUM_TaskLogBlockName.TASKLOG_Protect,RTInfo.Task,'write',[curBattery;threshBattery;0;0;0;]); % 更新log缓存
    |         printComInfo('[BatteryLife] RunOut',1)
    |     end
    | else
    |     sl = 1;
    | end
  function flag = isHeightLowerThanSwitchHeight_HoverUp:
    | function flag = isHeightLowerThanSwitchHeight_HoverUp
    | % 在盘旋上升模式判断高度过低
    | persistent duration
    | if isempty(duration)
    |     duration = 0;
    | end
    | modeCond = PathModeOut.flightTaskMode == ENUM_FlightTaskMode.HoverUpMode;
    | flag = false;
    | if modeCond && ...
    |         isUavInFix && ...
